simulink model "kinovaMicoSimscapeModel"  (R2021b)
settings: Solver=VariableStepAuto  StartTime=0.0  StopTime=0.3  FixedStep=0.01  RelTol=1e-3
PostLoadFcn:
  | micoRigidBodyTreeCreation;
  | IC=deg2rad([-90,180,180,0,0,0]);
  | interactiveHomePosition=deg2rad([-90 90 177.5 90 0 0]');
  | load("./KinovaMicoSimscapeVariantConfigurations.mat");
values from neighbouring files (symbols this model uses):
  micoCandlePosition = deg2rad([0,180,180,0,0,0])    [KinovaMicoSimscapeInitializeScript.m]    (also in generatingRandomTrajectory.m)
  ViaPointsTaskSpace = [ViaPointsTaskSpace;[[pi;0;pi],[pi;0;pi],[pi;0;pi],[pi;0;pi],[0;0;0],[0;0;0],[pi;0;pi]]]    [KinovaMicoSimscapeInitializeScript.m]    (also in generatingRandomTrajectory.m = [ViaPointsTaskSpace;zeros(3,7)])
undefined symbols (not defined in the file or in its folder): Mico, ViaPointsJointSpace, X, Y, Z
libraries: sm_lib x26, nesl_utility x19, robotcorelib x4, robotmaniplib x3, pid_lib x2
(part 32 of 50)

== matlab function kinovaMicoSimscapeModel/Variant Subsystem/TaskSpaceController/HybridImpedanceVelocityControl/Hybrid Impedance Velocity Control ==
  data: q input; dq input; ddq input; qd input; dqd input; torque output; ddqd input; f input; H input; C input; G input; test output
function [torque,test]     = ImpedanceVelocityControl(q,dq,ddq,qd,dqd,ddqd,f,H,C,G)
%% Joint Space variables
q1 = q(1);
q2 = q(2);
q3 = q(3);
q4 = q(4);
q5 = q(5);
q6 = q(6);

qd1 = qd(1);
qd2 = qd(2);
qd3 = qd(3);
qd4 = qd(4);
qd5 = qd(5);
qd6 = qd(6);


dq1 = qd(1);
dq2 = qd(2);
dq3 = qd(3);
dq4 = qd(4);
dq5 = qd(5);
dq6 = qd(6);


%% Define the Jacobian
jac=[(37*cos(q1)*cos(q4))/1000 - (7*cos(q1))/1000 - (29*sin(q1)*sin(q2))/100 - (37*cos(q5)*(cos(q1)*cos(q4) - sin(q4)*(sin(q1)*sin(q2)*sin(q3) + cos(q2)*cos(q3)*sin(q1))))/2000 + (37*sin(q5)*(cos(q1)*sin(q4) + cos(q4)*(sin(q1)*sin(q2)*sin(q3) + cos(q2)*cos(q3)*sin(q1))))/1000 - (29*3^(1/2)*((cos(q5)*(cos(q1)*cos(q4) - sin(q4)*(sin(q1)*sin(q2)*sin(q3) + cos(q2)*cos(q3)*sin(q1))))/2 - sin(q5)*(cos(q1)*sin(q4) + cos(q4)*(sin(q1)*sin(q2)*sin(q3) + cos(q2)*cos(q3)*sin(q1))) + (3^(1/2)*cos(q5)*(cos(q2)*sin(q1)*sin(q3) - cos(q3)*sin(q1)*sin(q2)))/2))/625 - (37*sin(q4)*(sin(q1)*sin(q2)*sin(q3) + cos(q2)*cos(q3)*sin(q1)))/1000 + (221*3^(1/2)*(cos(q1)*cos(q4) - sin(q4)*(sin(q1)*sin(q2)*sin(q3) + cos(q2)*cos(q3)*sin(q1))))/4000 - (37*3^(1/2)*cos(q5)*(cos(q2)*sin(q1)*sin(q3) - cos(q3)*sin(q1)*sin(q2)))/2000 - (4849*cos(q2)*sin(q1)*sin(q3))/20000 + (4849*cos(q3)*sin(q1)*sin(q2))/20000, (29*cos(q1)*cos(q2))/100 + (37*sin(q4)*(cos(q1)*cos(q2)*sin(q3) - cos(q1)*cos(q3)*sin(q2)))/1000 - (29*3^(1/2)*(cos(q4)*sin(q5)*(cos(q1)*cos(q2)*sin(q3) - cos(q1)*cos(q3)*sin(q2)) + (cos(q5)*sin(q4)*(cos(q1)*cos(q2)*sin(q3) - cos(q1)*cos(q3)*sin(q2)))/2 + (3^(1/2)*cos(q5)*(cos(q1)*cos(q2)*cos(q3) + cos(q1)*sin(q2)*sin(q3)))/2))/625 - (37*cos(q4)*sin(q5)*(cos(q1)*cos(q2)*sin(q3) - cos(q1)*cos(q3)*sin(q2)))/1000 - (37*cos(q5)*sin(q4)*(cos(q1)*cos(q2)*sin(q3) - cos(q1)*cos(q3)*sin(q2)))/2000 - (37*3^(1/2)*cos(q5)*(cos(q1)*cos(q2)*cos(q3) + cos(q1)*sin(q2)*sin(q3)))/2000 + (221*3^(1/2)*sin(q4)*(cos(q1)*cos(q2)*sin(q3) - cos(q1)*cos(q3)*sin(q2)))/4000 - (4849*cos(q1)*cos(q2)*cos(q3))/20000 - (4849*cos(q1)*sin(q2)*sin(q3))/20000, (29*3^(1/2)*(cos(q4)*sin(q5)*(cos(q1)*cos(q2)*sin(q3) - cos(q1)*cos(q3)*sin(q2)) + (cos(q5)*sin(q4)*(cos(q1)*cos(q2)*sin(q3) - cos(q1)*cos(q3)*sin(q2)))/2 + (3^(1/2)*cos(q5)*(cos(q1)*cos(q2)*cos(q3) + cos(q1)*sin(q2)*sin(q3)))/2))/625 - (37*sin(q4)*(cos(q1)*cos(q2)*sin(q3) - cos(q1)*cos(q3)*sin(q2)))/1000 + (37*cos(q4)*sin(q5)*(cos(q1)*cos(q2)*sin(q3) - cos(q1)*cos(q3)*sin(q2)))/1000 + (37*cos(q5)*sin(q4)*(cos(q1)*cos(q2)*sin(q3) - cos(q1)*cos(q3)*sin(q2)))/2000 + (37*3^(1/2)*cos(q5)*(cos(q1)*cos(q2)*cos(q3) + cos(q1)*sin(q2)*sin(q3)))/2000 - (221*3^(1/2)*sin(q4)*(cos(q1)*cos(q2)*sin(q3) - cos(q1)*cos(q3)*sin(q2)))/4000 + (4849*cos(q1)*cos(q2)*cos(q3))/20000 + (4849*cos(q1)*sin(q2)*sin(q3))/20000, (37*cos(q5)*(sin(q1)*sin(q4) - cos(q4)*(cos(q1)*cos(q2)*cos(q3) + cos(q1)*sin(q2)*sin(q3))))/2000 - (37*sin(q1)*sin(q4))/1000 + (37*sin(q5)*(cos(q4)*sin(q1) + sin(q4)*(cos(q1)*cos(q2)*cos(q3) + cos(q1)*sin(q2)*sin(q3))))/1000 + (37*cos(q4)*(cos(q1)*cos(q2)*cos(q3) + cos(q1)*sin(q2)*sin(q3)))/1000 + (29*3^(1/2)*((cos(q5)*(sin(q1)*sin(q4) - cos(q4)*(cos(q1)*cos(q2)*cos(q3) + cos(q1)*sin(q2)*sin(q3))))/2 + sin(q5)*(cos(q4)*sin(q1) + sin(q4)*(cos(q1)*cos(q2)*cos(q3) + cos(q1)*sin(q2)*sin(q3)))))/625 - (221*3^(1/2)*(sin(q1)*sin(q4) - cos(q4)*(cos(q1)*cos(q2)*cos(q3) + cos(q1)*sin(q2)*sin(q3))))/4000, (37*cos(q5)*(sin(q1)*sin(q4) - cos(q4)*(cos(q1)*cos(q2)*cos(q3) + cos(q1)*sin(q2)*sin(q3))))/1000 + (37*sin(q5)*(cos(q4)*sin(q1) + sin(q4)*(cos(q1)*cos(q2)*cos(q3) + cos(q1)*sin(q2)*sin(q3))))/2000 + (29*3^(1/2)*(cos(q5)*(sin(q1)*sin(q4) - cos(q4)*(cos(q1)*cos(q2)*cos(q3) + cos(q1)*sin(q2)*sin(q3))) + (sin(q5)*(cos(q4)*sin(q1) + sin(q4)*(cos(q1)*cos(q2)*cos(q3) + cos(q1)*sin(q2)*sin(q3))))/2 - (3^(1/2)*sin(q5)*(cos(q1)*cos(q2)*sin(q3) - cos(q1)*cos(q3)*sin(q2)))/2))/625 - (37*3^(1/2)*sin(q5)*(cos(q1)*cos(q2)*sin(q3) - cos(q1)*cos(q3)*sin(q2)))/2000,                                                                                                                                                                                                                                                                                                                                                                                                                                       0;
(7*sin(q1))/1000 - (29*cos(q1)*sin(q2))/100 - (37*cos(q4)*sin(q1))/1000 + (37*cos(q5)*(cos(q4)*sin(q1) + sin(q4)*(cos(q1)*cos(q2)*cos(q3) + cos(q1)*sin(q2)*sin(q3))))/2000 - (37*sin(q5)*(sin(q1)*sin(q4) - cos(q4)*(cos(q1)*cos(q2)*cos(q3) + cos(q1)*sin(q2)*sin(q3))))/1000 - (29*3^(1/2)*(sin(q5)*(sin(q1)*sin(q4) - cos(q4)*(cos(q1)*cos(q2)*cos(q3) + cos(q1)*sin(q2)*sin(q3))) - (cos(q5)*(cos(q4)*sin(q1) + sin(q4)*(cos(q1)*cos(q2)*cos(q3) + cos(q1)*sin(q2)*sin(q3))))/2 + (3^(1/2)*cos(q5)*(cos(q1)*cos(q2)*sin(q3) - cos(q1)*cos(q3)*sin(q2)))/2))/625 - (37*sin(q4)*(cos(q1)*cos(q2)*cos(q3) + cos(q1)*sin(q2)*sin(q3)))/1000 - (221*3^(1/2)*(cos(q4)*sin(q1) + sin(q4)*(cos(q1)*cos(q2)*cos(q3) + cos(q1)*sin(q2)*sin(q3))))/4000 - (37*3^(1/2)*cos(q5)*(cos(q1)*cos(q2)*sin(q3) - cos(q1)*cos(q3)*sin(q2)))/2000 - (4849*cos(q1)*cos(q2)*sin(q3))/20000 + (4849*cos(q1)*cos(q3)*sin(q2))/20000, (29*3^(1/2)*(cos(q4)*sin(q5)*(cos(q2)*sin(q1)*sin(q3) - cos(q3)*sin(q1)*sin(q2)) + (cos(q5)*sin(q4)*(cos(q2)*sin(q1)*sin(q3) - cos(q3)*sin(q1)*sin(q2)))/2 + (3^(1/2)*cos(q5)*(sin(q1)*sin(q2)*sin(q3) + cos(q2)*cos(q3)*sin(q1)))/2))/625 - (37*sin(q4)*(cos(q2)*sin(q1)*sin(q3) - cos(q3)*sin(q1)*sin(q2)))/1000 - (29*cos(q2)*sin(q1))/100 + (4849*sin(q1)*sin(q2)*sin(q3))/20000 + (37*cos(q4)*sin(q5)*(cos(q2)*sin(q1)*sin(q3) - cos(q3)*sin(q1)*sin(q2)))/1000 + (37*cos(q5)*sin(q4)*(cos(q2)*sin(q1)*sin(q3) - cos(q3)*sin(q1)*sin(q2)))/2000 + (37*3^(1/2)*cos(q5)*(sin(q1)*sin(q2)*sin(q3) + cos(q2)*cos(q3)*sin(q1)))/2000 + (4849*cos(q2)*cos(q3)*sin(q1))/20000 - (221*3^(1/2)*sin(q4)*(cos(q2)*sin(q1)*sin(q3) - cos(q3)*sin(q1)*sin(q2)))/4000, (37*sin(q4)*(cos(q2)*sin(q1)*sin(q3) - cos(q3)*sin(q1)*sin(q2)))/1000 - (29*3^(1/2)*(cos(q4)*sin(q5)*(cos(q2)*sin(q1)*sin(q3) - cos(q3)*sin(q1)*sin(q2)) + (cos(q5)*sin(q4)*(cos(q2)*sin(q1)*sin(q3) - cos(q3)*sin(q1)*sin(q2)))/2 + (3^(1/2)*cos(q5)*(sin(q1)*sin(q2)*sin(q3) + cos(q2)*cos(q3)*sin(q1)))/2))/625 - (4849*sin(q1)*sin(q2)*sin(q3))/20000 - (37*cos(q4)*sin(q5)*(cos(q2)*sin(q1)*sin(q3) - cos(q3)*sin(q1)*sin(q2)))/1000 - (37*cos(q5)*sin(q4)*(cos(q2)*sin(q1)*sin(q3) - cos(q3)*sin(q1)*sin(q2)))/2000 - (37*3^(1/2)*cos(q5)*(sin(q1)*sin(q2)*sin(q3) + cos(q2)*cos(q3)*sin(q1)))/2000 - (4849*cos(q2)*cos(q3)*sin(q1))/20000 + (221*3^(1/2)*sin(q4)*(cos(q2)*sin(q1)*sin(q3) - cos(q3)*sin(q1)*sin(q2)))/4000, (37*cos(q5)*(cos(q1)*sin(q4) + cos(q4)*(sin(q1)*sin(q2)*sin(q3) + cos(q2)*cos(q3)*sin(q1))))/2000 - (37*cos(q1)*sin(q4))/1000 + (37*sin(q5)*(cos(q1)*cos(q4) - sin(q4)*(sin(q1)*sin(q2)*sin(q3) + cos(q2)*cos(q3)*sin(q1))))/1000 - (37*cos(q4)*(sin(q1)*sin(q2)*sin(q3) + cos(q2)*cos(q3)*sin(q1)))/1000 + (29*3^(1/2)*((cos(q5)*(cos(q1)*sin(q4) + cos(q4)*(sin(q1)*sin(q2)*sin(q3) + cos(q2)*cos(q3)*sin(q1))))/2 + sin(q5)*(cos(q1)*cos(q4) - sin(q4)*(sin(q1)*sin(q2)*sin(q3) + cos(q2)*cos(q3)*sin(q1)))))/625 - (221*3^(1/2)*(cos(q1)*sin(q4) + cos(q4)*(sin(q1)*sin(q2)*sin(q3) + cos(q2)*cos(q3)*sin(q1))))/4000, (37*cos(q5)*(cos(q1)*sin(q4) + cos(q4)*(sin(q1)*sin(q2)*sin(q3) + cos(q2)*cos(q3)*sin(q1))))/1000 + (37*sin(q5)*(cos(q1)*cos(q4) - sin(q4)*(sin(q1)*sin(q2)*sin(q3) + cos(q2)*cos(q3)*sin(q1))))/2000 + (29*3^(1/2)*(cos(q5)*(cos(q1)*sin(q4) + cos(q4)*(sin(q1)*sin(q2)*sin(q3) + cos(q2)*cos(q3)*sin(q1))) + (sin(q5)*(cos(q1)*cos(q4) - sin(q4)*(sin(q1)*sin(q2)*sin(q3) + cos(q2)*cos(q3)*sin(q1))))/2 + (3^(1/2)*sin(q5)*(cos(q2)*sin(q1)*sin(q3) - cos(q3)*sin(q1)*sin(q2)))/2))/625 + (37*3^(1/2)*sin(q5)*(cos(q2)*sin(q1)*sin(q3) - cos(q3)*sin(q1)*sin(q2)))/2000,                                                                                                                                                                                                                                                                                                                                                                                                                                       0;
                                                                                                                                                                                                                                                                                                                                                                                                                                                                                                                                                                                                                                                                                                                                                                                                                                                                                                              0,                                                                                                                                                         (29*sin(q2))/100 + (4849*cos(q2)*sin(q3))/20000 - (4849*cos(q3)*sin(q2))/20000 - (29*3^(1/2)*(cos(q4)*sin(q5)*(cos(q2)*cos(q3) + sin(q2)*sin(q3)) - (3^(1/2)*cos(q5)*(cos(q2)*sin(q3) - cos(q3)*sin(q2)))/2 + (cos(q5)*sin(q4)*(cos(q2)*cos(q3) + sin(q2)*sin(q3)))/2))/625 + (37*sin(q4)*(cos(q2)*cos(q3) + sin(q2)*sin(q3)))/1000 + (37*3^(1/2)*cos(q5)*(cos(q2)*sin(q3) - cos(q3)*sin(q2)))/2000 + (221*3^(1/2)*sin(q4)*(cos(q2)*cos(q3) + sin(q2)*sin(q3)))/4000 - (37*cos(q4)*sin(q5)*(cos(q2)*cos(q3) + sin(q2)*sin(q3)))/1000 - (37*cos(q5)*sin(q4)*(cos(q2)*cos(q3) + sin(q2)*sin(q3)))/2000,                                                                                                                                                 (4849*cos(q3)*sin(q2))/20000 - (4849*cos(q2)*sin(q3))/20000 + (29*3^(1/2)*(cos(q4)*sin(q5)*(cos(q2)*cos(q3) + sin(q2)*sin(q3)) - (3^(1/2)*cos(q5)*(cos(q2)*sin(q3) - cos(q3)*sin(q2)))/2 + (cos(q5)*sin(q4)*(cos(q2)*cos(q3) + sin(q2)*sin(q3)))/2))/625 - (37*sin(q4)*(cos(q2)*cos(q3) + sin(q2)*sin(q3)))/1000 - (37*3^(1/2)*cos(q5)*(cos(q2)*sin(q3) - cos(q3)*sin(q2)))/2000 - (221*3^(1/2)*sin(q4)*(cos(q2)*cos(q3) + sin(q2)*sin(q3)))/4000 + (37*cos(q4)*sin(q5)*(cos(q2)*cos(q3) + sin(q2)*sin(q3)))/1000 + (37*cos(q5)*sin(q4)*(cos(q2)*cos(q3) + sin(q2)*sin(q3)))/2000,                                                                                                                                                                                                                                 (29*3^(1/2)*((cos(q4)*cos(q5)*(cos(q2)*sin(q3) - cos(q3)*sin(q2)))/2 - sin(q4)*sin(q5)*(cos(q2)*sin(q3) - cos(q3)*sin(q2))))/625 - (37*cos(q4)*(cos(q2)*sin(q3) - cos(q3)*sin(q2)))/1000 - (221*3^(1/2)*cos(q4)*(cos(q2)*sin(q3) - cos(q3)*sin(q2)))/4000 + (37*cos(q4)*cos(q5)*(cos(q2)*sin(q3) - cos(q3)*sin(q2)))/2000 - (37*sin(q4)*sin(q5)*(cos(q2)*sin(q3) - cos(q3)*sin(q2)))/1000,                                                                                                                                                                                 (37*cos(q4)*cos(q5)*(cos(q2)*sin(q3) - cos(q3)*sin(q2)))/1000 - (37*3^(1/2)*sin(q5)*(cos(q2)*cos(q3) + sin(q2)*sin(q3)))/2000 - (29*3^(1/2)*((3^(1/2)*sin(q5)*(cos(q2)*cos(q3) + sin(q2)*sin(q3)))/2 - cos(q4)*cos(q5)*(cos(q2)*sin(q3) - cos(q3)*sin(q2)) + (sin(q4)*sin(q5)*(cos(q2)*sin(q3) - cos(q3)*sin(q2)))/2))/625 - (37*sin(q4)*sin(q5)*(cos(q2)*sin(q3) - cos(q3)*sin(q2)))/2000,                                                                                                                                                                                                                                                                                                                                                                                                                                       0;
                                                                                                                                                                                                                                                                                                                                                                                                                                                                                                                                                                                                                                                                                                                                                                                                                                                                                                              0,                                                                                                                                                                                                                                                                                                                                                                                                                                                                                                                                                                                                                                                                                                                                                     -sin(q1),                                                                                                                                                                                                                                                                                                                                                                                                                                                                                                                                                                                                                                                                                                                           sin(q1),                                                                                                                                                                                                                                                                                                                                                                                                                                                                                                                                                                         cos(q1)*cos(q3)*sin(q2) - cos(q1)*cos(q2)*sin(q3),                                                                                                                                                                                                                                                                                                                                                                                                                    (cos(q1)*cos(q3)*sin(q2))/2 - (cos(q1)*cos(q2)*sin(q3))/2 - (3^(1/2)*(cos(q4)*sin(q1) + sin(q4)*(cos(q1)*cos(q2)*cos(q3) + cos(q1)*sin(q2)*sin(q3))))/2, (cos(q1)*cos(q3)*sin(q2))/4 - (3^(1/2)*(cos(q4)*sin(q1) + sin(q4)*(cos(q1)*cos(q2)*cos(q3) + cos(q1)*sin(q2)*sin(q3))))/4 - (cos(q1)*cos(q2)*sin(q3))/4 - (3^(1/2)*(sin(q5)*(sin(q1)*sin(q4) - cos(q4)*(cos(q1)*cos(q2)*cos(q3) + cos(q1)*sin(q2)*sin(q3))) - (cos(q5)*(cos(q4)*sin(q1) + sin(q4)*(cos(q1)*cos(q2)*cos(q3) + cos(q1)*sin(q2)*sin(q3))))/2 + (3^(1/2)*cos(q5)*(cos(q1)*cos(q2)*sin(q3) - cos(q1)*cos(q3)*sin(q2)))/2))/2;
                                                                                                                                                                                                                                                                                                                                                                                                                                                                                                                                                                                                                                                                                                                                                                                                                                                                                                              0,                                                                                                                                                                                                                                                                                                                                                                                                                                                                                                                                                                                                                                                                                                                                                     -cos(q1),                                                                                                                                                                                                                                                                                                                                                                                                                                                                                                                                                                                                                                                                                                                           cos(q1),                                                                                                                                                                                                                                                                                                                                                                                                                                                                                                                                                                         cos(q2)*sin(q1)*sin(q3) - cos(q3)*sin(q1)*sin(q2),                                                                                                                                                                                                                                                                                                                                                                                                                    (cos(q2)*sin(q1)*sin(q3))/2 - (3^(1/2)*(cos(q1)*cos(q4) - sin(q4)*(sin(q1)*sin(q2)*sin(q3) + cos(q2)*cos(q3)*sin(q1))))/2 - (cos(q3)*sin(q1)*sin(q2))/2, (3^(1/2)*((cos(q5)*(cos(q1)*cos(q4) - sin(q4)*(sin(q1)*sin(q2)*sin(q3) + cos(q2)*cos(q3)*sin(q1))))/2 - sin(q5)*(cos(q1)*sin(q4) + cos(q4)*(sin(q1)*sin(q2)*sin(q3) + cos(q2)*cos(q3)*sin(q1))) + (3^(1/2)*cos(q5)*(cos(q2)*sin(q1)*sin(q3) - cos(q3)*sin(q1)*sin(q2)))/2))/2 - (3^(1/2)*(cos(q1)*cos(q4) - sin(q4)*(sin(q1)*sin(q2)*sin(q3) + cos(q2)*cos(q3)*sin(q1))))/4 + (cos(q2)*sin(q1)*sin(q3))/4 - (cos(q3)*sin(q1)*sin(q2))/4;
                                                                                                                                                                                                                                                                                                                                                                                                                                                                                                                                                                                                                                                                                                                                                                                                                                                                                                             -1,                                                                                                                                                                                                                                                                                                                                                                                                                                                                                                                                                                                                                                                                                                                                                            0,                                                                                                                                                                                                                                                                                                                                                                                                                                                                                                                                                                                                                                                                                                                                 0,                                                                                                                                                                                                                                                                                                                                                                                                                                                                                                                                                                                       - cos(q2)*cos(q3) - sin(q2)*sin(q3),                                                                                                                                                                                                                                                                                                                                                                                                                                                                        (3^(1/2)*sin(q4)*(cos(q2)*sin(q3) - cos(q3)*sin(q2)))/2 - (sin(q2)*sin(q3))/2 - (cos(q2)*cos(q3))/2,                                                                                                                                             (3^(1/2)*sin(q4)*(cos(q2)*sin(q3) - cos(q3)*sin(q2)))/4 - (sin(q2)*sin(q3))/4 - (3^(1/2)*((3^(1/2)*cos(q5)*(cos(q2)*cos(q3) + sin(q2)*sin(q3)))/2 + cos(q4)*sin(q5)*(cos(q2)*sin(q3) - cos(q3)*sin(q2)) + (cos(q5)*sin(q4)*(cos(q2)*sin(q3) - cos(q3)*sin(q2)))/2))/2 - (cos(q2)*cos(q3))/4];
                        
%% Define the derivative of the jacobian
dJac=[(37*cos(q5)*(sin(q4)*(dq1*cos(q1)*cos(q2)*cos(q3) + dq1*cos(q1)*sin(q2)*sin(q3) + dq2*cos(q2)*sin(q1)*sin(q3) - dq2*cos(q3)*sin(q1)*sin(q2) - dq3*cos(q2)*sin(q1)*sin(q3) + dq3*cos(q3)*sin(q1)*sin(q2)) + dq1*cos(q4)*sin(q1) + dq4*cos(q1)*sin(q4) + dq4*cos(q4)*(sin(q1)*sin(q2)*sin(q3) + cos(q2)*cos(q3)*sin(q1))))/2000 + (37*sin(q5)*(cos(q4)*(dq1*cos(q1)*cos(q2)*cos(q3) + dq1*cos(q1)*sin(q2)*sin(q3) + dq2*cos(q2)*sin(q1)*sin(q3) - dq2*cos(q3)*sin(q1)*sin(q2) - dq3*cos(q2)*sin(q1)*sin(q3) + dq3*cos(q3)*sin(q1)*sin(q2)) - dq4*sin(q4)*(sin(q1)*sin(q2)*sin(q3) + cos(q2)*cos(q3)*sin(q1)) + dq4*cos(q1)*cos(q4) - dq1*sin(q1)*sin(q4)))/1000 + (29*3^(1/2)*((cos(q5)*(sin(q4)*(dq1*cos(q1)*cos(q2)*cos(q3) + dq1*cos(q1)*sin(q2)*sin(q3) + dq2*cos(q2)*sin(q1)*sin(q3) - dq2*cos(q3)*sin(q1)*sin(q2) - dq3*cos(q2)*sin(q1)*sin(q3) + dq3*cos(q3)*sin(q1)*sin(q2)) + dq1*cos(q4)*sin(q1) + dq4*cos(q1)*sin(q4) + dq4*cos(q4)*(sin(q1)*sin(q2)*sin(q3) + cos(q2)*cos(q3)*sin(q1))))/2 + sin(q5)*(cos(q4)*(dq1*cos(q1)*cos(q2)*cos(q3) + dq1*cos(q1)*sin(q2)*sin(q3) + dq2*cos(q2)*sin(q1)*sin(q3) - dq2*cos(q3)*sin(q1)*sin(q2) - dq3*cos(q2)*sin(q1)*sin(q3) + dq3*cos(q3)*sin(q1)*sin(q2)) - dq4*sin(q4)*(sin(q1)*sin(q2)*sin(q3) + cos(q2)*cos(q3)*sin(q1)) + dq4*cos(q1)*cos(q4) - dq1*sin(q1)*sin(q4)) - (3^(1/2)*cos(q5)*(dq1*cos(q1)*cos(q2)*sin(q3) - dq1*cos(q1)*cos(q3)*sin(q2) - dq2*cos(q2)*cos(q3)*sin(q1) + dq3*cos(q2)*cos(q3)*sin(q1) - dq2*sin(q1)*sin(q2)*sin(q3) + dq3*sin(q1)*sin(q2)*sin(q3)))/2 + dq5*cos(q5)*(cos(q1)*sin(q4) + cos(q4)*(sin(q1)*sin(q2)*sin(q3) + cos(q2)*cos(q3)*sin(q1))) + (dq5*sin(q5)*(cos(q1)*cos(q4) - sin(q4)*(sin(q1)*sin(q2)*sin(q3) + cos(q2)*cos(q3)*sin(q1))))/2 + (3^(1/2)*dq5*sin(q5)*(cos(q2)*sin(q1)*sin(q3) - cos(q3)*sin(q1)*sin(q2)))/2))/625 + (7*dq1*sin(q1))/1000 - (37*sin(q4)*(dq1*cos(q1)*cos(q2)*cos(q3) + dq1*cos(q1)*sin(q2)*sin(q3) + dq2*cos(q2)*sin(q1)*sin(q3) - dq2*cos(q3)*sin(q1)*sin(q2) - dq3*cos(q2)*sin(q1)*sin(q3) + dq3*cos(q3)*sin(q1)*sin(q2)))/1000 - (221*3^(1/2)*(sin(q4)*(dq1*cos(q1)*cos(q2)*cos(q3) + dq1*cos(q1)*sin(q2)*sin(q3) + dq2*cos(q2)*sin(q1)*sin(q3) - dq2*cos(q3)*sin(q1)*sin(q2) - dq3*cos(q2)*sin(q1)*sin(q3) + dq3*cos(q3)*sin(q1)*sin(q2)) + dq1*cos(q4)*sin(q1) + dq4*cos(q1)*sin(q4) + dq4*cos(q4)*(sin(q1)*sin(q2)*sin(q3) + cos(q2)*cos(q3)*sin(q1))))/4000 - (37*3^(1/2)*cos(q5)*(dq1*cos(q1)*cos(q2)*sin(q3) - dq1*cos(q1)*cos(q3)*sin(q2) - dq2*cos(q2)*cos(q3)*sin(q1) + dq3*cos(q2)*cos(q3)*sin(q1) - dq2*sin(q1)*sin(q2)*sin(q3) + dq3*sin(q1)*sin(q2)*sin(q3)))/2000 - (29*dq1*cos(q1)*sin(q2))/100 - (29*dq2*cos(q2)*sin(q1))/100 - (37*dq1*cos(q4)*sin(q1))/1000 - (37*dq4*cos(q1)*sin(q4))/1000 + (37*dq5*cos(q5)*(cos(q1)*sin(q4) + cos(q4)*(sin(q1)*sin(q2)*sin(q3) + cos(q2)*cos(q3)*sin(q1))))/1000 + (37*dq5*sin(q5)*(cos(q1)*cos(q4) - sin(q4)*(sin(q1)*sin(q2)*sin(q3) + cos(q2)*cos(q3)*sin(q1))))/2000 - (37*dq4*cos(q4)*(sin(q1)*sin(q2)*sin(q3) + cos(q2)*cos(q3)*sin(q1)))/1000 - (4849*dq1*cos(q1)*cos(q2)*sin(q3))/20000 + (4849*dq1*cos(q1)*cos(q3)*sin(q2))/20000 + (4849*dq2*cos(q2)*cos(q3)*sin(q1))/20000 - (4849*dq3*cos(q2)*cos(q3)*sin(q1))/20000 + (37*3^(1/2)*dq5*sin(q5)*(cos(q2)*sin(q1)*sin(q3) - cos(q3)*sin(q1)*sin(q2)))/2000 + (4849*dq2*sin(q1)*sin(q2)*sin(q3))/20000 - (4849*dq3*sin(q1)*sin(q2)*sin(q3))/20000, (29*3^(1/2)*(cos(q4)*sin(q5)*(dq2*cos(q1)*cos(q2)*cos(q3) - dq3*cos(q1)*cos(q2)*cos(q3) + dq1*cos(q2)*sin(q1)*sin(q3) - dq1*cos(q3)*sin(q1)*sin(q2) + dq2*cos(q1)*sin(q2)*sin(q3) - dq3*cos(q1)*sin(q2)*sin(q3)) + (cos(q5)*sin(q4)*(dq2*cos(q1)*cos(q2)*cos(q3) - dq3*cos(q1)*cos(q2)*cos(q3) + dq1*cos(q2)*sin(q1)*sin(q3) - dq1*cos(q3)*sin(q1)*sin(q2) + dq2*cos(q1)*sin(q2)*sin(q3) - dq3*cos(q1)*sin(q2)*sin(q3)))/2 + (3^(1/2)*cos(q5)*(dq1*cos(q2)*cos(q3)*sin(q1) - dq2*cos(q1)*cos(q2)*sin(q3) + dq2*cos(q1)*cos(q3)*sin(q2) + dq3*cos(q1)*cos(q2)*sin(q3) - dq3*cos(q1)*cos(q3)*sin(q2) + dq1*sin(q1)*sin(q2)*sin(q3)))/2 + (3^(1/2)*dq5*sin(q5)*(cos(q1)*cos(q2)*cos(q3) + cos(q1)*sin(q2)*sin(q3)))/2 - (dq4*cos(q4)*cos(q5)*(cos(q1)*cos(q2)*sin(q3) - cos(q1)*cos(q3)*sin(q2)))/2 - dq5*cos(q4)*cos(q5)*(cos(q1)*cos(q2)*sin(q3) - cos(q1)*cos(q3)*sin(q2)) + dq4*sin(q4)*sin(q5)*(cos(q1)*cos(q2)*sin(q3) - cos(q1)*cos(q3)*sin(q2)) + (dq5*sin(q4)*sin(q5)*(cos(q1)*cos(q2)*sin(q3) - cos(q1)*cos(q3)*sin(q2)))/2))/625 - (37*sin(q4)*(dq2*cos(q1)*cos(q2)*cos(q3) - dq3*cos(q1)*cos(q2)*cos(q3) + dq1*cos(q2)*sin(q1)*sin(q3) - dq1*cos(q3)*sin(q1)*sin(q2) + dq2*cos(q1)*sin(q2)*sin(q3) - dq3*cos(q1)*sin(q2)*sin(q3)))/1000 - (221*3^(1/2)*sin(q4)*(dq2*cos(q1)*cos(q2)*cos(q3) - dq3*cos(q1)*cos(q2)*cos(q3) + dq1*cos(q2)*sin(q1)*sin(q3) - dq1*cos(q3)*sin(q1)*sin(q2) + dq2*cos(q1)*sin(q2)*sin(q3) - dq3*cos(q1)*sin(q2)*sin(q3)))/4000 - (29*dq1*cos(q2)*sin(q1))/100 - (29*dq2*cos(q1)*sin(q2))/100 + (37*cos(q4)*sin(q5)*(dq2*cos(q1)*cos(q2)*cos(q3) - dq3*cos(q1)*cos(q2)*cos(q3) + dq1*cos(q2)*sin(q1)*sin(q3) - dq1*cos(q3)*sin(q1)*sin(q2) + dq2*cos(q1)*sin(q2)*sin(q3) - dq3*cos(q1)*sin(q2)*sin(q3)))/1000 + (37*cos(q5)*sin(q4)*(dq2*cos(q1)*cos(q2)*cos(q3) - dq3*cos(q1)*cos(q2)*cos(q3) + dq1*cos(q2)*sin(q1)*sin(q3) - dq1*cos(q3)*sin(q1)*sin(q2) + dq2*cos(q1)*sin(q2)*sin(q3) - dq3*cos(q1)*sin(q2)*sin(q3)))/2000 + (37*dq4*cos(q4)*(cos(q1)*cos(q2)*sin(q3) - cos(q1)*cos(q3)*sin(q2)))/1000 + (37*3^(1/2)*cos(q5)*(dq1*cos(q2)*cos(q3)*sin(q1) - dq2*cos(q1)*cos(q2)*sin(q3) + dq2*cos(q1)*cos(q3)*sin(q2) + dq3*cos(q1)*cos(q2)*sin(q3) - dq3*cos(q1)*cos(q3)*sin(q2) + dq1*sin(q1)*sin(q2)*sin(q3)))/2000 + (221*3^(1/2)*dq4*cos(q4)*(cos(q1)*cos(q2)*sin(q3) - cos(q1)*cos(q3)*sin(q2)))/4000 + (37*3^(1/2)*dq5*sin(q5)*(cos(q1)*cos(q2)*cos(q3) + cos(q1)*sin(q2)*sin(q3)))/2000 + (4849*dq1*cos(q2)*cos(q3)*sin(q1))/20000 - (4849*dq2*cos(q1)*cos(q2)*sin(q3))/20000 + (4849*dq2*cos(q1)*cos(q3)*sin(q2))/20000 + (4849*dq3*cos(q1)*cos(q2)*sin(q3))/20000 - (4849*dq3*cos(q1)*cos(q3)*sin(q2))/20000 + (4849*dq1*sin(q1)*sin(q2)*sin(q3))/20000 - (37*dq4*cos(q4)*cos(q5)*(cos(q1)*cos(q2)*sin(q3) - cos(q1)*cos(q3)*sin(q2)))/2000 - (37*dq5*cos(q4)*cos(q5)*(cos(q1)*cos(q2)*sin(q3) - cos(q1)*cos(q3)*sin(q2)))/1000 + (37*dq4*sin(q4)*sin(q5)*(cos(q1)*cos(q2)*sin(q3) - cos(q1)*cos(q3)*sin(q2)))/1000 + (37*dq5*sin(q4)*sin(q5)*(cos(q1)*cos(q2)*sin(q3) - cos(q1)*cos(q3)*sin(q2)))/2000, (37*sin(q4)*(dq2*cos(q1)*cos(q2)*cos(q3) - dq3*cos(q1)*cos(q2)*cos(q3) + dq1*cos(q2)*sin(q1)*sin(q3) - dq1*cos(q3)*sin(q1)*sin(q2) + dq2*cos(q1)*sin(q2)*sin(q3) - dq3*cos(q1)*sin(q2)*sin(q3)))/1000 - (29*3^(1/2)*(cos(q4)*sin(q5)*(dq2*cos(q1)*cos(q2)*cos(q3) - dq3*cos(q1)*cos(q2)*cos(q3) + dq1*cos(q2)*sin(q1)*sin(q3) - dq1*cos(q3)*sin(q1)*sin(q2) + dq2*cos(q1)*sin(q2)*sin(q3) - dq3*cos(q1)*sin(q2)*sin(q3)) + (cos(q5)*sin(q4)*(dq2*cos(q1)*cos(q2)*cos(q3) - dq3*cos(q1)*cos(q2)*cos(q3) + dq1*cos(q2)*sin(q1)*sin(q3) - dq1*cos(q3)*sin(q1)*sin(q2) + dq2*cos(q1)*sin(q2)*sin(q3) - dq3*cos(q1)*sin(q2)*sin(q3)))/2 + (3^(1/2)*cos(q5)*(dq1*cos(q2)*cos(q3)*sin(q1) - dq2*cos(q1)*cos(q2)*sin(q3) + dq2*cos(q1)*cos(q3)*sin(q2) + dq3*cos(q1)*cos(q2)*sin(q3) - dq3*cos(q1)*cos(q3)*sin(q2) + dq1*sin(q1)*sin(q2)*sin(q3)))/2 + (3^(1/2)*dq5*sin(q5)*(cos(q1)*cos(q2)*cos(q3) + cos(q1)*sin(q2)*sin(q3)))/2 - (dq4*cos(q4)*cos(q5)*(cos(q1)*cos(q2)*sin(q3) - cos(q1)*cos(q3)*sin(q2)))/2 - dq5*cos(q4)*cos(q5)*(cos(q1)*cos(q2)*sin(q3) - cos(q1)*cos(q3)*sin(q2)) + dq4*sin(q4)*sin(q5)*(cos(q1)*cos(q2)*sin(q3) - cos(q1)*cos(q3)*sin(q2)) + (dq5*sin(q4)*sin(q5)*(cos(q1)*cos(q2)*sin(q3) - cos(q1)*cos(q3)*sin(q2)))/2))/625 + (221*3^(1/2)*sin(q4)*(dq2*cos(q1)*cos(q2)*cos(q3) - dq3*cos(q1)*cos(q2)*cos(q3) + dq1*cos(q2)*sin(q1)*sin(q3) - dq1*cos(q3)*sin(q1)*sin(q2) + dq2*cos(q1)*sin(q2)*sin(q3) - dq3*cos(q1)*sin(q2)*sin(q3)))/4000 - (37*cos(q4)*sin(q5)*(dq2*cos(q1)*cos(q2)*cos(q3) - dq3*cos(q1)*cos(q2)*cos(q3) + dq1*cos(q2)*sin(q1)*sin(q3) - dq1*cos(q3)*sin(q1)*sin(q2) + dq2*cos(q1)*sin(q2)*sin(q3) - dq3*cos(q1)*sin(q2)*sin(q3)))/1000 - (37*cos(q5)*sin(q4)*(dq2*cos(q1)*cos(q2)*cos(q3) - dq3*cos(q1)*cos(q2)*cos(q3) + dq1*cos(q2)*sin(q1)*sin(q3) - dq1*cos(q3)*sin(q1)*sin(q2) + dq2*cos(q1)*sin(q2)*sin(q3) - dq3*cos(q1)*sin(q2)*sin(q3)))/2000 - (37*dq4*cos(q4)*(cos(q1)*cos(q2)*sin(q3) - cos(q1)*cos(q3)*sin(q2)))/1000 - (37*3^(1/2)*cos(q5)*(dq1*cos(q2)*cos(q3)*sin(q1) - dq2*cos(q1)*cos(q2)*sin(q3) + dq2*cos(q1)*cos(q3)*sin(q2) + dq3*cos(q1)*cos(q2)*sin(q3) - dq3*cos(q1)*cos(q3)*sin(q2) + dq1*sin(q1)*sin(q2)*sin(q3)))/2000 - (221*3^(1/2)*dq4*cos(q4)*(cos(q1)*cos(q2)*sin(q3) - cos(q1)*cos(q3)*sin(q2)))/4000 - (37*3^(1/2)*dq5*sin(q5)*(cos(q1)*cos(q2)*cos(q3) + cos(q1)*sin(q2)*sin(q3)))/2000 - (4849*dq1*cos(q2)*cos(q3)*sin(q1))/20000 + (4849*dq2*cos(q1)*cos(q2)*sin(q3))/20000 - (4849*dq2*cos(q1)*cos(q3)*sin(q2))/20000 - (4849*dq3*cos(q1)*cos(q2)*sin(q3))/20000 + (4849*dq3*cos(q1)*cos(q3)*sin(q2))/20000 - (4849*dq1*sin(q1)*sin(q2)*sin(q3))/20000 + (37*dq4*cos(q4)*cos(q5)*(cos(q1)*cos(q2)*sin(q3) - cos(q1)*cos(q3)*sin(q2)))/2000 + (37*dq5*cos(q4)*cos(q5)*(cos(q1)*cos(q2)*sin(q3) - cos(q1)*cos(q3)*sin(q2)))/1000 - (37*dq4*sin(q4)*sin(q5)*(cos(q1)*cos(q2)*sin(q3) - cos(q1)*cos(q3)*sin(q2)))/1000 - (37*dq5*sin(q4)*sin(q5)*(cos(q1)*cos(q2)*sin(q3) - cos(q1)*cos(q3)*sin(q2)))/2000, (37*cos(q5)*(cos(q4)*(dq1*cos(q2)*cos(q3)*sin(q1) - dq2*cos(q1)*cos(q2)*sin(q3) + dq2*cos(q1)*cos(q3)*sin(q2) + dq3*cos(q1)*cos(q2)*sin(q3) - dq3*cos(q1)*cos(q3)*sin(q2) + dq1*sin(q1)*sin(q2)*sin(q3)) + dq1*cos(q1)*sin(q4) + dq4*cos(q4)*sin(q1) + dq4*sin(q4)*(cos(q1)*cos(q2)*cos(q3) + cos(q1)*sin(q2)*sin(q3))))/2000 - (37*sin(q5)*(sin(q4)*(dq1*cos(q2)*cos(q3)*sin(q1) - dq2*cos(q1)*cos(q2)*sin(q3) + dq2*cos(q1)*cos(q3)*sin(q2) + dq3*cos(q1)*cos(q2)*sin(q3) - dq3*cos(q1)*cos(q3)*sin(q2) + dq1*sin(q1)*sin(q2)*sin(q3)) - dq1*cos(q1)*cos(q4) + dq4*sin(q1)*sin(q4) - dq4*cos(q4)*(cos(q1)*cos(q2)*cos(q3) + cos(q1)*sin(q2)*sin(q3))))/1000 + (29*3^(1/2)*((cos(q5)*(cos(q4)*(dq1*cos(q2)*cos(q3)*sin(q1) - dq2*cos(q1)*cos(q2)*sin(q3) + dq2*cos(q1)*cos(q3)*sin(q2) + dq3*cos(q1)*cos(q2)*sin(q3) - dq3*cos(q1)*cos(q3)*sin(q2) + dq1*sin(q1)*sin(q2)*sin(q3)) + dq1*cos(q1)*sin(q4) + dq4*cos(q4)*sin(q1) + dq4*sin(q4)*(cos(q1)*cos(q2)*cos(q3) + cos(q1)*sin(q2)*sin(q3))))/2 - sin(q5)*(sin(q4)*(dq1*cos(q2)*cos(q3)*sin(q1) - dq2*cos(q1)*cos(q2)*sin(q3) + dq2*cos(q1)*cos(q3)*sin(q2) + dq3*cos(q1)*cos(q2)*sin(q3) - dq3*cos(q1)*cos(q3)*sin(q2) + dq1*sin(q1)*sin(q2)*sin(q3)) - dq1*cos(q1)*cos(q4) + dq4*sin(q1)*sin(q4) - dq4*cos(q4)*(cos(q1)*cos(q2)*cos(q3) + cos(q1)*sin(q2)*sin(q3))) + dq5*cos(q5)*(cos(q4)*sin(q1) + sin(q4)*(cos(q1)*cos(q2)*cos(q3) + cos(q1)*sin(q2)*sin(q3))) - (dq5*sin(q5)*(sin(q1)*sin(q4) - cos(q4)*(cos(q1)*cos(q2)*cos(q3) + cos(q1)*sin(q2)*sin(q3))))/2))/625 - (221*3^(1/2)*(cos(q4)*(dq1*cos(q2)*cos(q3)*sin(q1) - dq2*cos(q1)*cos(q2)*sin(q3) + dq2*cos(q1)*cos(q3)*sin(q2) + dq3*cos(q1)*cos(q2)*sin(q3) - dq3*cos(q1)*cos(q3)*sin(q2) + dq1*sin(q1)*sin(q2)*sin(q3)) + dq1*cos(q1)*sin(q4) + dq4*cos(q4)*sin(q1) + dq4*sin(q4)*(cos(q1)*cos(q2)*cos(q3) + cos(q1)*sin(q2)*sin(q3))))/4000 - (37*cos(q4)*(dq1*cos(q2)*cos(q3)*sin(q1) - dq2*cos(q1)*cos(q2)*sin(q3) + dq2*cos(q1)*cos(q3)*sin(q2) + dq3*cos(q1)*cos(q2)*sin(q3) - dq3*cos(q1)*cos(q3)*sin(q2) + dq1*sin(q1)*sin(q2)*sin(q3)))/1000 - (37*dq1*cos(q1)*sin(q4))/1000 - (37*dq4*cos(q4)*sin(q1))/1000 + (37*dq5*cos(q5)*(cos(q4)*sin(q1) + sin(q4)*(cos(q1)*cos(q2)*cos(q3) + cos(q1)*sin(q2)*sin(q3))))/1000 - (37*dq5*sin(q5)*(sin(q1)*sin(q4) - cos(q4)*(cos(q1)*cos(q2)*cos(q3) + cos(q1)*sin(q2)*sin(q3))))/2000 - (37*dq4*sin(q4)*(cos(q1)*cos(q2)*cos(q3) + cos(q1)*sin(q2)*sin(q3)))/1000, (37*cos(q5)*(cos(q4)*(dq1*cos(q2)*cos(q3)*sin(q1) - dq2*cos(q1)*cos(q2)*sin(q3) + dq2*cos(q1)*cos(q3)*sin(q2) + dq3*cos(q1)*cos(q2)*sin(q3) - dq3*cos(q1)*cos(q3)*sin(q2) + dq1*sin(q1)*sin(q2)*sin(q3)) + dq1*cos(q1)*sin(q4) + dq4*cos(q4)*sin(q1) + dq4*sin(q4)*(cos(q1)*cos(q2)*cos(q3) + cos(q1)*sin(q2)*sin(q3))))/1000 - (37*sin(q5)*(sin(q4)*(dq1*cos(q2)*cos(q3)*sin(q1) - dq2*cos(q1)*cos(q2)*sin(q3) + dq2*cos(q1)*cos(q3)*sin(q2) + dq3*cos(q1)*cos(q2)*sin(q3) - dq3*cos(q1)*cos(q3)*sin(q2) + dq1*sin(q1)*sin(q2)*sin(q3)) - dq1*cos(q1)*cos(q4) + dq4*sin(q1)*sin(q4) - dq4*cos(q4)*(cos(q1)*cos(q2)*cos(q3) + cos(q1)*sin(q2)*sin(q3))))/2000 + (29*3^(1/2)*(cos(q5)*(cos(q4)*(dq1*cos(q2)*cos(q3)*sin(q1) - dq2*cos(q1)*cos(q2)*sin(q3) + dq2*cos(q1)*cos(q3)*sin(q2) + dq3*cos(q1)*cos(q2)*sin(q3) - dq3*cos(q1)*cos(q3)*sin(q2) + dq1*sin(q1)*sin(q2)*sin(q3)) + dq1*cos(q1)*sin(q4) + dq4*cos(q4)*sin(q1) + dq4*sin(q4)*(cos(q1)*cos(q2)*cos(q3) + cos(q1)*sin(q2)*sin(q3))) - (sin(q5)*(sin(q4)*(dq1*cos(q2)*cos(q3)*sin(q1) - dq2*cos(q1)*cos(q2)*sin(q3) + dq2*cos(q1)*cos(q3)*sin(q2) + dq3*cos(q1)*cos(q2)*sin(q3) - dq3*cos(q1)*cos(q3)*sin(q2) + dq1*sin(q1)*sin(q2)*sin(q3)) - dq1*cos(q1)*cos(q4) + dq4*sin(q1)*sin(q4) - dq4*cos(q4)*(cos(q1)*cos(q2)*cos(q3) + cos(q1)*sin(q2)*sin(q3))))/2 + (3^(1/2)*sin(q5)*(dq2*cos(q1)*cos(q2)*cos(q3) - dq3*cos(q1)*cos(q2)*cos(q3) + dq1*cos(q2)*sin(q1)*sin(q3) - dq1*cos(q3)*sin(q1)*sin(q2) + dq2*cos(q1)*sin(q2)*sin(q3) - dq3*cos(q1)*sin(q2)*sin(q3)))/2 + (dq5*cos(q5)*(cos(q4)*sin(q1) + sin(q4)*(cos(q1)*cos(q2)*cos(q3) + cos(q1)*sin(q2)*sin(q3))))/2 - dq5*sin(q5)*(sin(q1)*sin(q4) - cos(q4)*(cos(q1)*cos(q2)*cos(q3) + cos(q1)*sin(q2)*sin(q3))) - (3^(1/2)*dq5*cos(q5)*(cos(q1)*cos(q2)*sin(q3) - cos(q1)*cos(q3)*sin(q2)))/2))/625 + (37*3^(1/2)*sin(q5)*(dq2*cos(q1)*cos(q2)*cos(q3) - dq3*cos(q1)*cos(q2)*cos(q3) + dq1*cos(q2)*sin(q1)*sin(q3) - dq1*cos(q3)*sin(q1)*sin(q2) + dq2*cos(q1)*sin(q2)*sin(q3) - dq3*cos(q1)*sin(q2)*sin(q3)))/2000 + (37*dq5*cos(q5)*(cos(q4)*sin(q1) + sin(q4)*(cos(q1)*cos(q2)*cos(q3) + cos(q1)*sin(q2)*sin(q3))))/2000 - (37*dq5*sin(q5)*(sin(q1)*sin(q4) - cos(q4)*(cos(q1)*cos(q2)*cos(q3) + cos(q1)*sin(q2)*sin(q3))))/1000 - (37*3^(1/2)*dq5*cos(q5)*(cos(q1)*cos(q2)*sin(q3) - cos(q1)*cos(q3)*sin(q2)))/2000,                                                                                                                                                                                                                                                                                                                                                                                                                                                                                                                                                                                                                                                                                                                                                                                                                                                                                                                                                                                                                                                                                                                                                                                                                                                                                                                                                                                                                                                                                                                                                                                                                                                                                         0;
(221*3^(1/2)*(sin(q4)*(dq1*cos(q2)*cos(q3)*sin(q1) - dq2*cos(q1)*cos(q2)*sin(q3) + dq2*cos(q1)*cos(q3)*sin(q2) + dq3*cos(q1)*cos(q2)*sin(q3) - dq3*cos(q1)*cos(q3)*sin(q2) + dq1*sin(q1)*sin(q2)*sin(q3)) - dq1*cos(q1)*cos(q4) + dq4*sin(q1)*sin(q4) - dq4*cos(q4)*(cos(q1)*cos(q2)*cos(q3) + cos(q1)*sin(q2)*sin(q3))))/4000 - (37*sin(q5)*(cos(q4)*(dq1*cos(q2)*cos(q3)*sin(q1) - dq2*cos(q1)*cos(q2)*sin(q3) + dq2*cos(q1)*cos(q3)*sin(q2) + dq3*cos(q1)*cos(q2)*sin(q3) - dq3*cos(q1)*cos(q3)*sin(q2) + dq1*sin(q1)*sin(q2)*sin(q3)) + dq1*cos(q1)*sin(q4) + dq4*cos(q4)*sin(q1) + dq4*sin(q4)*(cos(q1)*cos(q2)*cos(q3) + cos(q1)*sin(q2)*sin(q3))))/1000 - (37*cos(q5)*(sin(q4)*(dq1*cos(q2)*cos(q3)*sin(q1) - dq2*cos(q1)*cos(q2)*sin(q3) + dq2*cos(q1)*cos(q3)*sin(q2) + dq3*cos(q1)*cos(q2)*sin(q3) - dq3*cos(q1)*cos(q3)*sin(q2) + dq1*sin(q1)*sin(q2)*sin(q3)) - dq1*cos(q1)*cos(q4) + dq4*sin(q1)*sin(q4) - dq4*cos(q4)*(cos(q1)*cos(q2)*cos(q3) + cos(q1)*sin(q2)*sin(q3))))/2000 + (7*dq1*cos(q1))/1000 - (29*3^(1/2)*((cos(q5)*(sin(q4)*(dq1*cos(q2)*cos(q3)*sin(q1) - dq2*cos(q1)*cos(q2)*sin(q3) + dq2*cos(q1)*cos(q3)*sin(q2) + dq3*cos(q1)*cos(q2)*sin(q3) - dq3*cos(q1)*cos(q3)*sin(q2) + dq1*sin(q1)*sin(q2)*sin(q3)) - dq1*cos(q1)*cos(q4) + dq4*sin(q1)*sin(q4) - dq4*cos(q4)*(cos(q1)*cos(q2)*cos(q3) + cos(q1)*sin(q2)*sin(q3))))/2 + sin(q5)*(cos(q4)*(dq1*cos(q2)*cos(q3)*sin(q1) - dq2*cos(q1)*cos(q2)*sin(q3) + dq2*cos(q1)*cos(q3)*sin(q2) + dq3*cos(q1)*cos(q2)*sin(q3) - dq3*cos(q1)*cos(q3)*sin(q2) + dq1*sin(q1)*sin(q2)*sin(q3)) + dq1*cos(q1)*sin(q4) + dq4*cos(q4)*sin(q1) + dq4*sin(q4)*(cos(q1)*cos(q2)*cos(q3) + cos(q1)*sin(q2)*sin(q3))) + dq5*cos(q5)*(sin(q1)*sin(q4) - cos(q4)*(cos(q1)*cos(q2)*cos(q3) + cos(q1)*sin(q2)*sin(q3))) + (dq5*sin(q5)*(cos(q4)*sin(q1) + sin(q4)*(cos(q1)*cos(q2)*cos(q3) + cos(q1)*sin(q2)*sin(q3))))/2 - (3^(1/2)*cos(q5)*(dq2*cos(q1)*cos(q2)*cos(q3) - dq3*cos(q1)*cos(q2)*cos(q3) + dq1*cos(q2)*sin(q1)*sin(q3) - dq1*cos(q3)*sin(q1)*sin(q2) + dq2*cos(q1)*sin(q2)*sin(q3) - dq3*cos(q1)*sin(q2)*sin(q3)))/2 - (3^(1/2)*dq5*sin(q5)*(cos(q1)*cos(q2)*sin(q3) - cos(q1)*cos(q3)*sin(q2)))/2))/625 + (37*sin(q4)*(dq1*cos(q2)*cos(q3)*sin(q1) - dq2*cos(q1)*cos(q2)*sin(q3) + dq2*cos(q1)*cos(q3)*sin(q2) + dq3*cos(q1)*cos(q2)*sin(q3) - dq3*cos(q1)*cos(q3)*sin(q2) + dq1*sin(q1)*sin(q2)*sin(q3)))/1000 - (29*dq2*cos(q1)*cos(q2))/100 - (37*dq1*cos(q1)*cos(q4))/1000 + (29*dq1*sin(q1)*sin(q2))/100 + (37*dq4*sin(q1)*sin(q4))/1000 - (37*dq5*cos(q5)*(sin(q1)*sin(q4) - cos(q4)*(cos(q1)*cos(q2)*cos(q3) + cos(q1)*sin(q2)*sin(q3))))/1000 - (37*dq5*sin(q5)*(cos(q4)*sin(q1) + sin(q4)*(cos(q1)*cos(q2)*cos(q3) + cos(q1)*sin(q2)*sin(q3))))/2000 - (37*dq4*cos(q4)*(cos(q1)*cos(q2)*cos(q3) + cos(q1)*sin(q2)*sin(q3)))/1000 + (37*3^(1/2)*cos(q5)*(dq2*cos(q1)*cos(q2)*cos(q3) - dq3*cos(q1)*cos(q2)*cos(q3) + dq1*cos(q2)*sin(q1)*sin(q3) - dq1*cos(q3)*sin(q1)*sin(q2) + dq2*cos(q1)*sin(q2)*sin(q3) - dq3*cos(q1)*sin(q2)*sin(q3)))/2000 + (37*3^(1/2)*dq5*sin(q5)*(cos(q1)*cos(q2)*sin(q3) - cos(q1)*cos(q3)*sin(q2)))/2000 + (4849*dq2*cos(q1)*cos(q2)*cos(q3))/20000 - (4849*dq3*cos(q1)*cos(q2)*cos(q3))/20000 + (4849*dq1*cos(q2)*sin(q1)*sin(q3))/20000 - (4849*dq1*cos(q3)*sin(q1)*sin(q2))/20000 + (4849*dq2*cos(q1)*sin(q2)*sin(q3))/20000 - (4849*dq3*cos(q1)*sin(q2)*sin(q3))/20000, (29*3^(1/2)*((3^(1/2)*cos(q5)*(dq1*cos(q1)*cos(q2)*cos(q3) + dq1*cos(q1)*sin(q2)*sin(q3) + dq2*cos(q2)*sin(q1)*sin(q3) - dq2*cos(q3)*sin(q1)*sin(q2) - dq3*cos(q2)*sin(q1)*sin(q3) + dq3*cos(q3)*sin(q1)*sin(q2)))/2 + cos(q4)*sin(q5)*(dq1*cos(q1)*cos(q2)*sin(q3) - dq1*cos(q1)*cos(q3)*sin(q2) - dq2*cos(q2)*cos(q3)*sin(q1) + dq3*cos(q2)*cos(q3)*sin(q1) - dq2*sin(q1)*sin(q2)*sin(q3) + dq3*sin(q1)*sin(q2)*sin(q3)) + (cos(q5)*sin(q4)*(dq1*cos(q1)*cos(q2)*sin(q3) - dq1*cos(q1)*cos(q3)*sin(q2) - dq2*cos(q2)*cos(q3)*sin(q1) + dq3*cos(q2)*cos(q3)*sin(q1) - dq2*sin(q1)*sin(q2)*sin(q3) + dq3*sin(q1)*sin(q2)*sin(q3)))/2 - (3^(1/2)*dq5*sin(q5)*(sin(q1)*sin(q2)*sin(q3) + cos(q2)*cos(q3)*sin(q1)))/2 + (dq4*cos(q4)*cos(q5)*(cos(q2)*sin(q1)*sin(q3) - cos(q3)*sin(q1)*sin(q2)))/2 + dq5*cos(q4)*cos(q5)*(cos(q2)*sin(q1)*sin(q3) - cos(q3)*sin(q1)*sin(q2)) - dq4*sin(q4)*sin(q5)*(cos(q2)*sin(q1)*sin(q3) - cos(q3)*sin(q1)*sin(q2)) - (dq5*sin(q4)*sin(q5)*(cos(q2)*sin(q1)*sin(q3) - cos(q3)*sin(q1)*sin(q2)))/2))/625 - (37*sin(q4)*(dq1*cos(q1)*cos(q2)*sin(q3) - dq1*cos(q1)*cos(q3)*sin(q2) - dq2*cos(q2)*cos(q3)*sin(q1) + dq3*cos(q2)*cos(q3)*sin(q1) - dq2*sin(q1)*sin(q2)*sin(q3) + dq3*sin(q1)*sin(q2)*sin(q3)))/1000 + (37*3^(1/2)*cos(q5)*(dq1*cos(q1)*cos(q2)*cos(q3) + dq1*cos(q1)*sin(q2)*sin(q3) + dq2*cos(q2)*sin(q1)*sin(q3) - dq2*cos(q3)*sin(q1)*sin(q2) - dq3*cos(q2)*sin(q1)*sin(q3) + dq3*cos(q3)*sin(q1)*sin(q2)))/2000 - (221*3^(1/2)*sin(q4)*(dq1*cos(q1)*cos(q2)*sin(q3) - dq1*cos(q1)*cos(q3)*sin(q2) - dq2*cos(q2)*cos(q3)*sin(q1) + dq3*cos(q2)*cos(q3)*sin(q1) - dq2*sin(q1)*sin(q2)*sin(q3) + dq3*sin(q1)*sin(q2)*sin(q3)))/4000 - (29*dq1*cos(q1)*cos(q2))/100 + (29*dq2*sin(q1)*sin(q2))/100 + (37*cos(q4)*sin(q5)*(dq1*cos(q1)*cos(q2)*sin(q3) - dq1*cos(q1)*cos(q3)*sin(q2) - dq2*cos(q2)*cos(q3)*sin(q1) + dq3*cos(q2)*cos(q3)*sin(q1) - dq2*sin(q1)*sin(q2)*sin(q3) + dq3*sin(q1)*sin(q2)*sin(q3)))/1000 + (37*cos(q5)*sin(q4)*(dq1*cos(q1)*cos(q2)*sin(q3) - dq1*cos(q1)*cos(q3)*sin(q2) - dq2*cos(q2)*cos(q3)*sin(q1) + dq3*cos(q2)*cos(q3)*sin(q1) - dq2*sin(q1)*sin(q2)*sin(q3) + dq3*sin(q1)*sin(q2)*sin(q3)))/2000 - (37*dq4*cos(q4)*(cos(q2)*sin(q1)*sin(q3) - cos(q3)*sin(q1)*sin(q2)))/1000 + (4849*dq1*cos(q1)*cos(q2)*cos(q3))/20000 - (221*3^(1/2)*dq4*cos(q4)*(cos(q2)*sin(q1)*sin(q3) - cos(q3)*sin(q1)*sin(q2)))/4000 - (37*3^(1/2)*dq5*sin(q5)*(sin(q1)*sin(q2)*sin(q3) + cos(q2)*cos(q3)*sin(q1)))/2000 + (4849*dq1*cos(q1)*sin(q2)*sin(q3))/20000 + (4849*dq2*cos(q2)*sin(q1)*sin(q3))/20000 - (4849*dq2*cos(q3)*sin(q1)*sin(q2))/20000 - (4849*dq3*cos(q2)*sin(q1)*sin(q3))/20000 + (4849*dq3*cos(q3)*sin(q1)*sin(q2))/20000 + (37*dq4*cos(q4)*cos(q5)*(cos(q2)*sin(q1)*sin(q3) - cos(q3)*sin(q1)*sin(q2)))/2000 + (37*dq5*cos(q4)*cos(q5)*(cos(q2)*sin(q1)*sin(q3) - cos(q3)*sin(q1)*sin(q2)))/1000 - (37*dq4*sin(q4)*sin(q5)*(cos(q2)*sin(q1)*sin(q3) - cos(q3)*sin(q1)*sin(q2)))/1000 - (37*dq5*sin(q4)*sin(q5)*(cos(q2)*sin(q1)*sin(q3) - cos(q3)*sin(q1)*sin(q2)))/2000, (37*sin(q4)*(dq1*cos(q1)*cos(q2)*sin(q3) - dq1*cos(q1)*cos(q3)*sin(q2) - dq2*cos(q2)*cos(q3)*sin(q1) + dq3*cos(q2)*cos(q3)*sin(q1) - dq2*sin(q1)*sin(q2)*sin(q3) + dq3*sin(q1)*sin(q2)*sin(q3)))/1000 - (29*3^(1/2)*((3^(1/2)*cos(q5)*(dq1*cos(q1)*cos(q2)*cos(q3) + dq1*cos(q1)*sin(q2)*sin(q3) + dq2*cos(q2)*sin(q1)*sin(q3) - dq2*cos(q3)*sin(q1)*sin(q2) - dq3*cos(q2)*sin(q1)*sin(q3) + dq3*cos(q3)*sin(q1)*sin(q2)))/2 + cos(q4)*sin(q5)*(dq1*cos(q1)*cos(q2)*sin(q3) - dq1*cos(q1)*cos(q3)*sin(q2) - dq2*cos(q2)*cos(q3)*sin(q1) + dq3*cos(q2)*cos(q3)*sin(q1) - dq2*sin(q1)*sin(q2)*sin(q3) + dq3*sin(q1)*sin(q2)*sin(q3)) + (cos(q5)*sin(q4)*(dq1*cos(q1)*cos(q2)*sin(q3) - dq1*cos(q1)*cos(q3)*sin(q2) - dq2*cos(q2)*cos(q3)*sin(q1) + dq3*cos(q2)*cos(q3)*sin(q1) - dq2*sin(q1)*sin(q2)*sin(q3) + dq3*sin(q1)*sin(q2)*sin(q3)))/2 - (3^(1/2)*dq5*sin(q5)*(sin(q1)*sin(q2)*sin(q3) + cos(q2)*cos(q3)*sin(q1)))/2 + (dq4*cos(q4)*cos(q5)*(cos(q2)*sin(q1)*sin(q3) - cos(q3)*sin(q1)*sin(q2)))/2 + dq5*cos(q4)*cos(q5)*(cos(q2)*sin(q1)*sin(q3) - cos(q3)*sin(q1)*sin(q2)) - dq4*sin(q4)*sin(q5)*(cos(q2)*sin(q1)*sin(q3) - cos(q3)*sin(q1)*sin(q2)) - (dq5*sin(q4)*sin(q5)*(cos(q2)*sin(q1)*sin(q3) - cos(q3)*sin(q1)*sin(q2)))/2))/625 - (37*3^(1/2)*cos(q5)*(dq1*cos(q1)*cos(q2)*cos(q3) + dq1*cos(q1)*sin(q2)*sin(q3) + dq2*cos(q2)*sin(q1)*sin(q3) - dq2*cos(q3)*sin(q1)*sin(q2) - dq3*cos(q2)*sin(q1)*sin(q3) + dq3*cos(q3)*sin(q1)*sin(q2)))/2000 + (221*3^(1/2)*sin(q4)*(dq1*cos(q1)*cos(q2)*sin(q3) - dq1*cos(q1)*cos(q3)*sin(q2) - dq2*cos(q2)*cos(q3)*sin(q1) + dq3*cos(q2)*cos(q3)*sin(q1) - dq2*sin(q1)*sin(q2)*sin(q3) + dq3*sin(q1)*sin(q2)*sin(q3)))/4000 - (37*cos(q4)*sin(q5)*(dq1*cos(q1)*cos(q2)*sin(q3) - dq1*cos(q1)*cos(q3)*sin(q2) - dq2*cos(q2)*cos(q3)*sin(q1) + dq3*cos(q2)*cos(q3)*sin(q1) - dq2*sin(q1)*sin(q2)*sin(q3) + dq3*sin(q1)*sin(q2)*sin(q3)))/1000 - (37*cos(q5)*sin(q4)*(dq1*cos(q1)*cos(q2)*sin(q3) - dq1*cos(q1)*cos(q3)*sin(q2) - dq2*cos(q2)*cos(q3)*sin(q1) + dq3*cos(q2)*cos(q3)*sin(q1) - dq2*sin(q1)*sin(q2)*sin(q3) + dq3*sin(q1)*sin(q2)*sin(q3)))/2000 + (37*dq4*cos(q4)*(cos(q2)*sin(q1)*sin(q3) - cos(q3)*sin(q1)*sin(q2)))/1000 - (4849*dq1*cos(q1)*cos(q2)*cos(q3))/20000 + (221*3^(1/2)*dq4*cos(q4)*(cos(q2)*sin(q1)*sin(q3) - cos(q3)*sin(q1)*sin(q2)))/4000 + (37*3^(1/2)*dq5*sin(q5)*(sin(q1)*sin(q2)*sin(q3) + cos(q2)*cos(q3)*sin(q1)))/2000 - (4849*dq1*cos(q1)*sin(q2)*sin(q3))/20000 - (4849*dq2*cos(q2)*sin(q1)*sin(q3))/20000 + (4849*dq2*cos(q3)*sin(q1)*sin(q2))/20000 + (4849*dq3*cos(q2)*sin(q1)*sin(q3))/20000 - (4849*dq3*cos(q3)*sin(q1)*sin(q2))/20000 - (37*dq4*cos(q4)*cos(q5)*(cos(q2)*sin(q1)*sin(q3) - cos(q3)*sin(q1)*sin(q2)))/2000 - (37*dq5*cos(q4)*cos(q5)*(cos(q2)*sin(q1)*sin(q3) - cos(q3)*sin(q1)*sin(q2)))/1000 + (37*dq4*sin(q4)*sin(q5)*(cos(q2)*sin(q1)*sin(q3) - cos(q3)*sin(q1)*sin(q2)))/1000 + (37*dq5*sin(q4)*sin(q5)*(cos(q2)*sin(q1)*sin(q3) - cos(q3)*sin(q1)*sin(q2)))/2000, (29*3^(1/2)*((cos(q5)*(cos(q4)*(dq1*cos(q1)*cos(q2)*cos(q3) + dq1*cos(q1)*sin(q2)*sin(q3) + dq2*cos(q2)*sin(q1)*sin(q3) - dq2*cos(q3)*sin(q1)*sin(q2) - dq3*cos(q2)*sin(q1)*sin(q3) + dq3*cos(q3)*sin(q1)*sin(q2)) - dq4*sin(q4)*(sin(q1)*sin(q2)*sin(q3) + cos(q2)*cos(q3)*sin(q1)) + dq4*cos(q1)*cos(q4) - dq1*sin(q1)*sin(q4)))/2 - sin(q5)*(sin(q4)*(dq1*cos(q1)*cos(q2)*cos(q3) + dq1*cos(q1)*sin(q2)*sin(q3) + dq2*cos(q2)*sin(q1)*sin(q3) - dq2*cos(q3)*sin(q1)*sin(q2) - dq3*cos(q2)*sin(q1)*sin(q3) + dq3*cos(q3)*sin(q1)*sin(q2)) + dq1*cos(q4)*sin(q1) + dq4*cos(q1)*sin(q4) + dq4*cos(q4)*(sin(q1)*sin(q2)*sin(q3) + cos(q2)*cos(q3)*sin(q1))) + dq5*cos(q5)*(cos(q1)*cos(q4) - sin(q4)*(sin(q1)*sin(q2)*sin(q3) + cos(q2)*cos(q3)*sin(q1))) - (dq5*sin(q5)*(cos(q1)*sin(q4) + cos(q4)*(sin(q1)*sin(q2)*sin(q3) + cos(q2)*cos(q3)*sin(q1))))/2))/625 + (37*cos(q5)*(cos(q4)*(dq1*cos(q1)*cos(q2)*cos(q3) + dq1*cos(q1)*sin(q2)*sin(q3) + dq2*cos(q2)*sin(q1)*sin(q3) - dq2*cos(q3)*sin(q1)*sin(q2) - dq3*cos(q2)*sin(q1)*sin(q3) + dq3*cos(q3)*sin(q1)*sin(q2)) - dq4*sin(q4)*(sin(q1)*sin(q2)*sin(q3) + cos(q2)*cos(q3)*sin(q1)) + dq4*cos(q1)*cos(q4) - dq1*sin(q1)*sin(q4)))/2000 - (37*sin(q5)*(sin(q4)*(dq1*cos(q1)*cos(q2)*cos(q3) + dq1*cos(q1)*sin(q2)*sin(q3) + dq2*cos(q2)*sin(q1)*sin(q3) - dq2*cos(q3)*sin(q1)*sin(q2) - dq3*cos(q2)*sin(q1)*sin(q3) + dq3*cos(q3)*sin(q1)*sin(q2)) + dq1*cos(q4)*sin(q1) + dq4*cos(q1)*sin(q4) + dq4*cos(q4)*(sin(q1)*sin(q2)*sin(q3) + cos(q2)*cos(q3)*sin(q1))))/1000 - (37*cos(q4)*(dq1*cos(q1)*cos(q2)*cos(q3) + dq1*cos(q1)*sin(q2)*sin(q3) + dq2*cos(q2)*sin(q1)*sin(q3) - dq2*cos(q3)*sin(q1)*sin(q2) - dq3*cos(q2)*sin(q1)*sin(q3) + dq3*cos(q3)*sin(q1)*sin(q2)))/1000 - (221*3^(1/2)*(cos(q4)*(dq1*cos(q1)*cos(q2)*cos(q3) + dq1*cos(q1)*sin(q2)*sin(q3) + dq2*cos(q2)*sin(q1)*sin(q3) - dq2*cos(q3)*sin(q1)*sin(q2) - dq3*cos(q2)*sin(q1)*sin(q3) + dq3*cos(q3)*sin(q1)*sin(q2)) - dq4*sin(q4)*(sin(q1)*sin(q2)*sin(q3) + cos(q2)*cos(q3)*sin(q1)) + dq4*cos(q1)*cos(q4) - dq1*sin(q1)*sin(q4)))/4000 + (37*dq4*sin(q4)*(sin(q1)*sin(q2)*sin(q3) + cos(q2)*cos(q3)*sin(q1)))/1000 - (37*dq4*cos(q1)*cos(q4))/1000 + (37*dq1*sin(q1)*sin(q4))/1000 + (37*dq5*cos(q5)*(cos(q1)*cos(q4) - sin(q4)*(sin(q1)*sin(q2)*sin(q3) + cos(q2)*cos(q3)*sin(q1))))/1000 - (37*dq5*sin(q5)*(cos(q1)*sin(q4) + cos(q4)*(sin(q1)*sin(q2)*sin(q3) + cos(q2)*cos(q3)*sin(q1))))/2000, (37*cos(q5)*(cos(q4)*(dq1*cos(q1)*cos(q2)*cos(q3) + dq1*cos(q1)*sin(q2)*sin(q3) + dq2*cos(q2)*sin(q1)*sin(q3) - dq2*cos(q3)*sin(q1)*sin(q2) - dq3*cos(q2)*sin(q1)*sin(q3) + dq3*cos(q3)*sin(q1)*sin(q2)) - dq4*sin(q4)*(sin(q1)*sin(q2)*sin(q3) + cos(q2)*cos(q3)*sin(q1)) + dq4*cos(q1)*cos(q4) - dq1*sin(q1)*sin(q4)))/1000 - (37*sin(q5)*(sin(q4)*(dq1*cos(q1)*cos(q2)*cos(q3) + dq1*cos(q1)*sin(q2)*sin(q3) + dq2*cos(q2)*sin(q1)*sin(q3) - dq2*cos(q3)*sin(q1)*sin(q2) - dq3*cos(q2)*sin(q1)*sin(q3) + dq3*cos(q3)*sin(q1)*sin(q2)) + dq1*cos(q4)*sin(q1) + dq4*cos(q1)*sin(q4) + dq4*cos(q4)*(sin(q1)*sin(q2)*sin(q3) + cos(q2)*cos(q3)*sin(q1))))/2000 + (29*3^(1/2)*(cos(q5)*(cos(q4)*(dq1*cos(q1)*cos(q2)*cos(q3) + dq1*cos(q1)*sin(q2)*sin(q3) + dq2*cos(q2)*sin(q1)*sin(q3) - dq2*cos(q3)*sin(q1)*sin(q2) - dq3*cos(q2)*sin(q1)*sin(q3) + dq3*cos(q3)*sin(q1)*sin(q2)) - dq4*sin(q4)*(sin(q1)*sin(q2)*sin(q3) + cos(q2)*cos(q3)*sin(q1)) + dq4*cos(q1)*cos(q4) - dq1*sin(q1)*sin(q4)) - (sin(q5)*(sin(q4)*(dq1*cos(q1)*cos(q2)*cos(q3) + dq1*cos(q1)*sin(q2)*sin(q3) + dq2*cos(q2)*sin(q1)*sin(q3) - dq2*cos(q3)*sin(q1)*sin(q2) - dq3*cos(q2)*sin(q1)*sin(q3) + dq3*cos(q3)*sin(q1)*sin(q2)) + dq1*cos(q4)*sin(q1) + dq4*cos(q1)*sin(q4) + dq4*cos(q4)*(sin(q1)*sin(q2)*sin(q3) + cos(q2)*cos(q3)*sin(q1))))/2 + (3^(1/2)*sin(q5)*(dq1*cos(q1)*cos(q2)*sin(q3) - dq1*cos(q1)*cos(q3)*sin(q2) - dq2*cos(q2)*cos(q3)*sin(q1) + dq3*cos(q2)*cos(q3)*sin(q1) - dq2*sin(q1)*sin(q2)*sin(q3) + dq3*sin(q1)*sin(q2)*sin(q3)))/2 + (dq5*cos(q5)*(cos(q1)*cos(q4) - sin(q4)*(sin(q1)*sin(q2)*sin(q3) + cos(q2)*cos(q3)*sin(q1))))/2 - dq5*sin(q5)*(cos(q1)*sin(q4) + cos(q4)*(sin(q1)*sin(q2)*sin(q3) + cos(q2)*cos(q3)*sin(q1))) + (3^(1/2)*dq5*cos(q5)*(cos(q2)*sin(q1)*sin(q3) - cos(q3)*sin(q1)*sin(q2)))/2))/625 + (37*3^(1/2)*sin(q5)*(dq1*cos(q1)*cos(q2)*sin(q3) - dq1*cos(q1)*cos(q3)*sin(q2) - dq2*cos(q2)*cos(q3)*sin(q1) + dq3*cos(q2)*cos(q3)*sin(q1) - dq2*sin(q1)*sin(q2)*sin(q3) + dq3*sin(q1)*sin(q2)*sin(q3)))/2000 + (37*dq5*cos(q5)*(cos(q1)*cos(q4) - sin(q4)*(sin(q1)*sin(q2)*sin(q3) + cos(q2)*cos(q3)*sin(q1))))/2000 - (37*dq5*sin(q5)*(cos(q1)*sin(q4) + cos(q4)*(sin(q1)*sin(q2)*sin(q3) + cos(q2)*cos(q3)*sin(q1))))/1000 + (37*3^(1/2)*dq5*cos(q5)*(cos(q2)*sin(q1)*sin(q3) - cos(q3)*sin(q1)*sin(q2)))/2000,                                                                                                                                                                                                                                                                                                                                                                                                                                                                                                                                                                                                                                                                                                                                                                                                                                                                                                                                                                                                                                                                                                                                                                                                                                                                                                                                                                                                                                                                                                                                                                                                                                                                                         0;
                                                                                                                                                                                                                                                                                                                                                                                                                                                                                                                                                                                                                                                                                                                                                                                                                                                                                                                                                                                                                                                                                                                                                                                                                                                                                                                                                                                                                                                                                                                                                                                                                                                                                                                                                                                                                                                                                                                                                                                                                                                                                                                                                                                                                                                                                                                                                                                                                                                                                                                                                                                                                                                                                                                                                                                                                                                                                                                                                                                                                                                                                                                                                                                                                                                                                                                                                                                       0,                                                                                                                                                                                                                                                                                                                                                                                                                                                                                                                                                                                                                                                                                                                                                                                                                                                                                                                                                                                                                                                                                                                              (37*sin(q4)*(dq2*cos(q2)*sin(q3) - dq2*cos(q3)*sin(q2) - dq3*cos(q2)*sin(q3) + dq3*cos(q3)*sin(q2)))/1000 + (29*dq2*cos(q2))/100 - (29*3^(1/2)*(cos(q4)*sin(q5)*(dq2*cos(q2)*sin(q3) - dq2*cos(q3)*sin(q2) - dq3*cos(q2)*sin(q3) + dq3*cos(q3)*sin(q2)) + (cos(q5)*sin(q4)*(dq2*cos(q2)*sin(q3) - dq2*cos(q3)*sin(q2) - dq3*cos(q2)*sin(q3) + dq3*cos(q3)*sin(q2)))/2 + (3^(1/2)*cos(q5)*(dq2*cos(q2)*cos(q3) - dq3*cos(q2)*cos(q3) + dq2*sin(q2)*sin(q3) - dq3*sin(q2)*sin(q3)))/2 - dq4*sin(q4)*sin(q5)*(cos(q2)*cos(q3) + sin(q2)*sin(q3)) - (dq5*sin(q4)*sin(q5)*(cos(q2)*cos(q3) + sin(q2)*sin(q3)))/2 + (3^(1/2)*dq5*sin(q5)*(cos(q2)*sin(q3) - cos(q3)*sin(q2)))/2 + (dq4*cos(q4)*cos(q5)*(cos(q2)*cos(q3) + sin(q2)*sin(q3)))/2 + dq5*cos(q4)*cos(q5)*(cos(q2)*cos(q3) + sin(q2)*sin(q3))))/625 + (37*dq4*cos(q4)*(cos(q2)*cos(q3) + sin(q2)*sin(q3)))/1000 - (37*cos(q4)*sin(q5)*(dq2*cos(q2)*sin(q3) - dq2*cos(q3)*sin(q2) - dq3*cos(q2)*sin(q3) + dq3*cos(q3)*sin(q2)))/1000 - (37*cos(q5)*sin(q4)*(dq2*cos(q2)*sin(q3) - dq2*cos(q3)*sin(q2) - dq3*cos(q2)*sin(q3) + dq3*cos(q3)*sin(q2)))/2000 - (4849*dq2*cos(q2)*cos(q3))/20000 + (4849*dq3*cos(q2)*cos(q3))/20000 - (4849*dq2*sin(q2)*sin(q3))/20000 + (4849*dq3*sin(q2)*sin(q3))/20000 - (37*3^(1/2)*cos(q5)*(dq2*cos(q2)*cos(q3) - dq3*cos(q2)*cos(q3) + dq2*sin(q2)*sin(q3) - dq3*sin(q2)*sin(q3)))/2000 + (221*3^(1/2)*sin(q4)*(dq2*cos(q2)*sin(q3) - dq2*cos(q3)*sin(q2) - dq3*cos(q2)*sin(q3) + dq3*cos(q3)*sin(q2)))/4000 + (37*dq4*sin(q4)*sin(q5)*(cos(q2)*cos(q3) + sin(q2)*sin(q3)))/1000 + (37*dq5*sin(q4)*sin(q5)*(cos(q2)*cos(q3) + sin(q2)*sin(q3)))/2000 + (221*3^(1/2)*dq4*cos(q4)*(cos(q2)*cos(q3) + sin(q2)*sin(q3)))/4000 - (37*3^(1/2)*dq5*sin(q5)*(cos(q2)*sin(q3) - cos(q3)*sin(q2)))/2000 - (37*dq4*cos(q4)*cos(q5)*(cos(q2)*cos(q3) + sin(q2)*sin(q3)))/2000 - (37*dq5*cos(q4)*cos(q5)*(cos(q2)*cos(q3) + sin(q2)*sin(q3)))/1000,                                                                                                                                                                                                                                                                                                                                                                                                                                                                                                                                                                                                                                                                                                                                                                                                                                                                                                                                                                                                                                                                                       (29*3^(1/2)*(cos(q4)*sin(q5)*(dq2*cos(q2)*sin(q3) - dq2*cos(q3)*sin(q2) - dq3*cos(q2)*sin(q3) + dq3*cos(q3)*sin(q2)) + (cos(q5)*sin(q4)*(dq2*cos(q2)*sin(q3) - dq2*cos(q3)*sin(q2) - dq3*cos(q2)*sin(q3) + dq3*cos(q3)*sin(q2)))/2 + (3^(1/2)*cos(q5)*(dq2*cos(q2)*cos(q3) - dq3*cos(q2)*cos(q3) + dq2*sin(q2)*sin(q3) - dq3*sin(q2)*sin(q3)))/2 - dq4*sin(q4)*sin(q5)*(cos(q2)*cos(q3) + sin(q2)*sin(q3)) - (dq5*sin(q4)*sin(q5)*(cos(q2)*cos(q3) + sin(q2)*sin(q3)))/2 + (3^(1/2)*dq5*sin(q5)*(cos(q2)*sin(q3) - cos(q3)*sin(q2)))/2 + (dq4*cos(q4)*cos(q5)*(cos(q2)*cos(q3) + sin(q2)*sin(q3)))/2 + dq5*cos(q4)*cos(q5)*(cos(q2)*cos(q3) + sin(q2)*sin(q3))))/625 - (37*sin(q4)*(dq2*cos(q2)*sin(q3) - dq2*cos(q3)*sin(q2) - dq3*cos(q2)*sin(q3) + dq3*cos(q3)*sin(q2)))/1000 - (37*dq4*cos(q4)*(cos(q2)*cos(q3) + sin(q2)*sin(q3)))/1000 + (37*cos(q4)*sin(q5)*(dq2*cos(q2)*sin(q3) - dq2*cos(q3)*sin(q2) - dq3*cos(q2)*sin(q3) + dq3*cos(q3)*sin(q2)))/1000 + (37*cos(q5)*sin(q4)*(dq2*cos(q2)*sin(q3) - dq2*cos(q3)*sin(q2) - dq3*cos(q2)*sin(q3) + dq3*cos(q3)*sin(q2)))/2000 + (4849*dq2*cos(q2)*cos(q3))/20000 - (4849*dq3*cos(q2)*cos(q3))/20000 + (4849*dq2*sin(q2)*sin(q3))/20000 - (4849*dq3*sin(q2)*sin(q3))/20000 + (37*3^(1/2)*cos(q5)*(dq2*cos(q2)*cos(q3) - dq3*cos(q2)*cos(q3) + dq2*sin(q2)*sin(q3) - dq3*sin(q2)*sin(q3)))/2000 - (221*3^(1/2)*sin(q4)*(dq2*cos(q2)*sin(q3) - dq2*cos(q3)*sin(q2) - dq3*cos(q2)*sin(q3) + dq3*cos(q3)*sin(q2)))/4000 - (37*dq4*sin(q4)*sin(q5)*(cos(q2)*cos(q3) + sin(q2)*sin(q3)))/1000 - (37*dq5*sin(q4)*sin(q5)*(cos(q2)*cos(q3) + sin(q2)*sin(q3)))/2000 - (221*3^(1/2)*dq4*cos(q4)*(cos(q2)*cos(q3) + sin(q2)*sin(q3)))/4000 + (37*3^(1/2)*dq5*sin(q5)*(cos(q2)*sin(q3) - cos(q3)*sin(q2)))/2000 + (37*dq4*cos(q4)*cos(q5)*(cos(q2)*cos(q3) + sin(q2)*sin(q3)))/2000 + (37*dq5*cos(q4)*cos(q5)*(cos(q2)*cos(q3) + sin(q2)*sin(q3)))/1000,                                                                                                                                                                                                                                                                                                                                                                                                                                                                                                                                                                                                                                                                                                                                                                                                                                                                                                                                                                                                                                                    (37*cos(q4)*(dq2*cos(q2)*cos(q3) - dq3*cos(q2)*cos(q3) + dq2*sin(q2)*sin(q3) - dq3*sin(q2)*sin(q3)))/1000 - (29*3^(1/2)*((cos(q4)*cos(q5)*(dq2*cos(q2)*cos(q3) - dq3*cos(q2)*cos(q3) + dq2*sin(q2)*sin(q3) - dq3*sin(q2)*sin(q3)))/2 - sin(q4)*sin(q5)*(dq2*cos(q2)*cos(q3) - dq3*cos(q2)*cos(q3) + dq2*sin(q2)*sin(q3) - dq3*sin(q2)*sin(q3)) + dq4*cos(q4)*sin(q5)*(cos(q2)*sin(q3) - cos(q3)*sin(q2)) + (dq4*cos(q5)*sin(q4)*(cos(q2)*sin(q3) - cos(q3)*sin(q2)))/2 + (dq5*cos(q4)*sin(q5)*(cos(q2)*sin(q3) - cos(q3)*sin(q2)))/2 + dq5*cos(q5)*sin(q4)*(cos(q2)*sin(q3) - cos(q3)*sin(q2))))/625 + (37*dq4*sin(q4)*(cos(q2)*sin(q3) - cos(q3)*sin(q2)))/1000 - (37*cos(q4)*cos(q5)*(dq2*cos(q2)*cos(q3) - dq3*cos(q2)*cos(q3) + dq2*sin(q2)*sin(q3) - dq3*sin(q2)*sin(q3)))/2000 + (37*sin(q4)*sin(q5)*(dq2*cos(q2)*cos(q3) - dq3*cos(q2)*cos(q3) + dq2*sin(q2)*sin(q3) - dq3*sin(q2)*sin(q3)))/1000 + (221*3^(1/2)*cos(q4)*(dq2*cos(q2)*cos(q3) - dq3*cos(q2)*cos(q3) + dq2*sin(q2)*sin(q3) - dq3*sin(q2)*sin(q3)))/4000 - (37*dq4*cos(q4)*sin(q5)*(cos(q2)*sin(q3) - cos(q3)*sin(q2)))/1000 - (37*dq4*cos(q5)*sin(q4)*(cos(q2)*sin(q3) - cos(q3)*sin(q2)))/2000 - (37*dq5*cos(q4)*sin(q5)*(cos(q2)*sin(q3) - cos(q3)*sin(q2)))/2000 - (37*dq5*cos(q5)*sin(q4)*(cos(q2)*sin(q3) - cos(q3)*sin(q2)))/1000 + (221*3^(1/2)*dq4*sin(q4)*(cos(q2)*sin(q3) - cos(q3)*sin(q2)))/4000,                                                                                                                                                                                                                                                                                                                                                                                                                                                                                                                                                                                                                                                                                                                                                                                                                                                                                                                                                         (37*sin(q4)*sin(q5)*(dq2*cos(q2)*cos(q3) - dq3*cos(q2)*cos(q3) + dq2*sin(q2)*sin(q3) - dq3*sin(q2)*sin(q3)))/2000 - (37*cos(q4)*cos(q5)*(dq2*cos(q2)*cos(q3) - dq3*cos(q2)*cos(q3) + dq2*sin(q2)*sin(q3) - dq3*sin(q2)*sin(q3)))/1000 - (29*3^(1/2)*(cos(q4)*cos(q5)*(dq2*cos(q2)*cos(q3) - dq3*cos(q2)*cos(q3) + dq2*sin(q2)*sin(q3) - dq3*sin(q2)*sin(q3)) - (sin(q4)*sin(q5)*(dq2*cos(q2)*cos(q3) - dq3*cos(q2)*cos(q3) + dq2*sin(q2)*sin(q3) - dq3*sin(q2)*sin(q3)))/2 + (3^(1/2)*sin(q5)*(dq2*cos(q2)*sin(q3) - dq2*cos(q3)*sin(q2) - dq3*cos(q2)*sin(q3) + dq3*cos(q3)*sin(q2)))/2 + (dq4*cos(q4)*sin(q5)*(cos(q2)*sin(q3) - cos(q3)*sin(q2)))/2 + dq4*cos(q5)*sin(q4)*(cos(q2)*sin(q3) - cos(q3)*sin(q2)) + dq5*cos(q4)*sin(q5)*(cos(q2)*sin(q3) - cos(q3)*sin(q2)) + (dq5*cos(q5)*sin(q4)*(cos(q2)*sin(q3) - cos(q3)*sin(q2)))/2 + (3^(1/2)*dq5*cos(q5)*(cos(q2)*cos(q3) + sin(q2)*sin(q3)))/2))/625 - (37*3^(1/2)*sin(q5)*(dq2*cos(q2)*sin(q3) - dq2*cos(q3)*sin(q2) - dq3*cos(q2)*sin(q3) + dq3*cos(q3)*sin(q2)))/2000 - (37*dq4*cos(q4)*sin(q5)*(cos(q2)*sin(q3) - cos(q3)*sin(q2)))/2000 - (37*dq4*cos(q5)*sin(q4)*(cos(q2)*sin(q3) - cos(q3)*sin(q2)))/1000 - (37*dq5*cos(q4)*sin(q5)*(cos(q2)*sin(q3) - cos(q3)*sin(q2)))/1000 - (37*dq5*cos(q5)*sin(q4)*(cos(q2)*sin(q3) - cos(q3)*sin(q2)))/2000 - (37*3^(1/2)*dq5*cos(q5)*(cos(q2)*cos(q3) + sin(q2)*sin(q3)))/2000,                                                                                                                                                                                                                                                                                                                                                                                                                                                                                                                                                                                                                                                                                                                                                                                                                                                                                                                                                                                                                                                                                                                                                                                                                                                                                                                                                                                                                                                                                                                                                                                                                                                                                         0;
                                                                                                                                                                                                                                                                                                                                                                                                                                                                                                                                                                                                                                                                                                                                                                                                                                                                                                                                                                                                                                                                                                                                                                                                                                                                                                                                                                                                                                                                                                                                                                                                                                                                                                                                                                                                                                                                                                                                                                                                                                                                                                                                                                                                                                                                                                                                                                                                                                                                                                                                                                                                                                                                                                                                                                                                                                                                                                                                                                                                                                                                                                                                                                                                                                                                                                                                                                                       0,                                                                                                                                                                                                                                                                                                                                                                                                                                                                                                                                                                                                                                                                                                                                                                                                                                                                                                                                                                                                                                                                                                                                                                                                                                                                                                                                                                                                                                                                                                                                                                                                                                                                                                                                                                                                                                                                                                                                                                                                                                                                                                                                                                                                                                                                                                                                                                                                                                                                                                                                                                                                                                                                                                                                                                                                                                                                                                                                                                                                                                           -dq1*cos(q1),                                                                                                                                                                                                                                                                                                                                                                                                                                                                                                                                                                                                                                                                                                                                                                                                                                                                                                                                                                                                                                                                                                                                                                                                                                                                                                                                                                                                                                                                                                                                                                                                                                                                                                                                                                                                                                                                                                                                                                                                                                                                                                                                                                                                                                                                                                                                                                                                                                                                                                                                                                                                                                                                                                                                                                                                                                                                                                                                                                              dq1*cos(q1),                                                                                                                                                                                                                                                                                                                                                                                                                                                                                                                                                                                                                                                                                                                                                                                                                                                                                                                                                                                                                                                                                                                                                                                                                                                                                                                                                                                                                                                                                                                                                                                                                                                                                                                                                                                                                                                                                                                                                                                                                                                                                                                                                                                                                                                     dq2*cos(q1)*cos(q2)*cos(q3) - dq3*cos(q1)*cos(q2)*cos(q3) + dq1*cos(q2)*sin(q1)*sin(q3) - dq1*cos(q3)*sin(q1)*sin(q2) + dq2*cos(q1)*sin(q2)*sin(q3) - dq3*cos(q1)*sin(q2)*sin(q3),                                                                                                                                                                                                                                                                                                                                                                                                                                                                                                                                                                                                                                                                                                                                                                                                                                                                                                                                                                                                                                                                                                                                                                                                                                                                                                                                                                                                                                                                                                                                                                                                                                                                                                                                                                                                          (3^(1/2)*(sin(q4)*(dq1*cos(q2)*cos(q3)*sin(q1) - dq2*cos(q1)*cos(q2)*sin(q3) + dq2*cos(q1)*cos(q3)*sin(q2) + dq3*cos(q1)*cos(q2)*sin(q3) - dq3*cos(q1)*cos(q3)*sin(q2) + dq1*sin(q1)*sin(q2)*sin(q3)) - dq1*cos(q1)*cos(q4) + dq4*sin(q1)*sin(q4) - dq4*cos(q4)*(cos(q1)*cos(q2)*cos(q3) + cos(q1)*sin(q2)*sin(q3))))/2 + (dq2*cos(q1)*cos(q2)*cos(q3))/2 - (dq3*cos(q1)*cos(q2)*cos(q3))/2 + (dq1*cos(q2)*sin(q1)*sin(q3))/2 - (dq1*cos(q3)*sin(q1)*sin(q2))/2 + (dq2*cos(q1)*sin(q2)*sin(q3))/2 - (dq3*cos(q1)*sin(q2)*sin(q3))/2, (3^(1/2)*(sin(q4)*(dq1*cos(q2)*cos(q3)*sin(q1) - dq2*cos(q1)*cos(q2)*sin(q3) + dq2*cos(q1)*cos(q3)*sin(q2) + dq3*cos(q1)*cos(q2)*sin(q3) - dq3*cos(q1)*cos(q3)*sin(q2) + dq1*sin(q1)*sin(q2)*sin(q3)) - dq1*cos(q1)*cos(q4) + dq4*sin(q1)*sin(q4) - dq4*cos(q4)*(cos(q1)*cos(q2)*cos(q3) + cos(q1)*sin(q2)*sin(q3))))/4 - (3^(1/2)*((cos(q5)*(sin(q4)*(dq1*cos(q2)*cos(q3)*sin(q1) - dq2*cos(q1)*cos(q2)*sin(q3) + dq2*cos(q1)*cos(q3)*sin(q2) + dq3*cos(q1)*cos(q2)*sin(q3) - dq3*cos(q1)*cos(q3)*sin(q2) + dq1*sin(q1)*sin(q2)*sin(q3)) - dq1*cos(q1)*cos(q4) + dq4*sin(q1)*sin(q4) - dq4*cos(q4)*(cos(q1)*cos(q2)*cos(q3) + cos(q1)*sin(q2)*sin(q3))))/2 + sin(q5)*(cos(q4)*(dq1*cos(q2)*cos(q3)*sin(q1) - dq2*cos(q1)*cos(q2)*sin(q3) + dq2*cos(q1)*cos(q3)*sin(q2) + dq3*cos(q1)*cos(q2)*sin(q3) - dq3*cos(q1)*cos(q3)*sin(q2) + dq1*sin(q1)*sin(q2)*sin(q3)) + dq1*cos(q1)*sin(q4) + dq4*cos(q4)*sin(q1) + dq4*sin(q4)*(cos(q1)*cos(q2)*cos(q3) + cos(q1)*sin(q2)*sin(q3))) + dq5*cos(q5)*(sin(q1)*sin(q4) - cos(q4)*(cos(q1)*cos(q2)*cos(q3) + cos(q1)*sin(q2)*sin(q3))) + (dq5*sin(q5)*(cos(q4)*sin(q1) + sin(q4)*(cos(q1)*cos(q2)*cos(q3) + cos(q1)*sin(q2)*sin(q3))))/2 - (3^(1/2)*cos(q5)*(dq2*cos(q1)*cos(q2)*cos(q3) - dq3*cos(q1)*cos(q2)*cos(q3) + dq1*cos(q2)*sin(q1)*sin(q3) - dq1*cos(q3)*sin(q1)*sin(q2) + dq2*cos(q1)*sin(q2)*sin(q3) - dq3*cos(q1)*sin(q2)*sin(q3)))/2 - (3^(1/2)*dq5*sin(q5)*(cos(q1)*cos(q2)*sin(q3) - cos(q1)*cos(q3)*sin(q2)))/2))/2 + (dq2*cos(q1)*cos(q2)*cos(q3))/4 - (dq3*cos(q1)*cos(q2)*cos(q3))/4 + (dq1*cos(q2)*sin(q1)*sin(q3))/4 - (dq1*cos(q3)*sin(q1)*sin(q2))/4 + (dq2*cos(q1)*sin(q2)*sin(q3))/4 - (dq3*cos(q1)*sin(q2)*sin(q3))/4;
                                                                                                                                                                                                                                                                                                                                                                                                                                                                                                                                                                                                                                                                                                                                                                                                                                                                                                                                                                                                                                                                                                                                                                                                                                                                                                                                                                                                                                                                                                                                                                                                                                                                                                                                                                                                                                                                                                                                                                                                                                                                                                                                                                                                                                                                                                                                                                                                                                                                                                                                                                                                                                                                                                                                                                                                                                                                                                                                                                                                                                                                                                                                                                                                                                                                                                                                                                                       0,                                                                                                                                                                                                                                                                                                                                                                                                                                                                                                                                                                                                                                                                                                                                                                                                                                                                                                                                                                                                                                                                                                                                                                                                                                                                                                                                                                                                                                                                                                                                                                                                                                                                                                                                                                                                                                                                                                                                                                                                                                                                                                                                                                                                                                                                                                                                                                                                                                                                                                                                                                                                                                                                                                                                                                                                                                                                                                                                                                                                                                            dq1*sin(q1),                                                                                                                                                                                                                                                                                                                                                                                                                                                                                                                                                                                                                                                                                                                                                                                                                                                                                                                                                                                                                                                                                                                                                                                                                                                                                                                                                                                                                                                                                                                                                                                                                                                                                                                                                                                                                                                                                                                                                                                                                                                                                                                                                                                                                                                                                                                                                                                                                                                                                                                                                                                                                                                                                                                                                                                                                                                                                                                                                                             -dq1*sin(q1),                                                                                                                                                                                                                                                                                                                                                                                                                                                                                                                                                                                                                                                                                                                                                                                                                                                                                                                                                                                                                                                                                                                                                                                                                                                                                                                                                                                                                                                                                                                                                                                                                                                                                                                                                                                                                                                                                                                                                                                                                                                                                                                                                                                                                                                     dq1*cos(q1)*cos(q2)*sin(q3) - dq1*cos(q1)*cos(q3)*sin(q2) - dq2*cos(q2)*cos(q3)*sin(q1) + dq3*cos(q2)*cos(q3)*sin(q1) - dq2*sin(q1)*sin(q2)*sin(q3) + dq3*sin(q1)*sin(q2)*sin(q3),                                                                                                                                                                                                                                                                                                                                                                                                                                                                                                                                                                                                                                                                                                                                                                                                                                                                                                                                                                                                                                                                                                                                                                                                                                                                                                                                                                                                                                                                                                                                                                                                                                                                                                                                                                                                          (3^(1/2)*(sin(q4)*(dq1*cos(q1)*cos(q2)*cos(q3) + dq1*cos(q1)*sin(q2)*sin(q3) + dq2*cos(q2)*sin(q1)*sin(q3) - dq2*cos(q3)*sin(q1)*sin(q2) - dq3*cos(q2)*sin(q1)*sin(q3) + dq3*cos(q3)*sin(q1)*sin(q2)) + dq1*cos(q4)*sin(q1) + dq4*cos(q1)*sin(q4) + dq4*cos(q4)*(sin(q1)*sin(q2)*sin(q3) + cos(q2)*cos(q3)*sin(q1))))/2 + (dq1*cos(q1)*cos(q2)*sin(q3))/2 - (dq1*cos(q1)*cos(q3)*sin(q2))/2 - (dq2*cos(q2)*cos(q3)*sin(q1))/2 + (dq3*cos(q2)*cos(q3)*sin(q1))/2 - (dq2*sin(q1)*sin(q2)*sin(q3))/2 + (dq3*sin(q1)*sin(q2)*sin(q3))/2, (3^(1/2)*(sin(q4)*(dq1*cos(q1)*cos(q2)*cos(q3) + dq1*cos(q1)*sin(q2)*sin(q3) + dq2*cos(q2)*sin(q1)*sin(q3) - dq2*cos(q3)*sin(q1)*sin(q2) - dq3*cos(q2)*sin(q1)*sin(q3) + dq3*cos(q3)*sin(q1)*sin(q2)) + dq1*cos(q4)*sin(q1) + dq4*cos(q1)*sin(q4) + dq4*cos(q4)*(sin(q1)*sin(q2)*sin(q3) + cos(q2)*cos(q3)*sin(q1))))/4 - (3^(1/2)*((cos(q5)*(sin(q4)*(dq1*cos(q1)*cos(q2)*cos(q3) + dq1*cos(q1)*sin(q2)*sin(q3) + dq2*cos(q2)*sin(q1)*sin(q3) - dq2*cos(q3)*sin(q1)*sin(q2) - dq3*cos(q2)*sin(q1)*sin(q3) + dq3*cos(q3)*sin(q1)*sin(q2)) + dq1*cos(q4)*sin(q1) + dq4*cos(q1)*sin(q4) + dq4*cos(q4)*(sin(q1)*sin(q2)*sin(q3) + cos(q2)*cos(q3)*sin(q1))))/2 + sin(q5)*(cos(q4)*(dq1*cos(q1)*cos(q2)*cos(q3) + dq1*cos(q1)*sin(q2)*sin(q3) + dq2*cos(q2)*sin(q1)*sin(q3) - dq2*cos(q3)*sin(q1)*sin(q2) - dq3*cos(q2)*sin(q1)*sin(q3) + dq3*cos(q3)*sin(q1)*sin(q2)) - dq4*sin(q4)*(sin(q1)*sin(q2)*sin(q3) + cos(q2)*cos(q3)*sin(q1)) + dq4*cos(q1)*cos(q4) - dq1*sin(q1)*sin(q4)) - (3^(1/2)*cos(q5)*(dq1*cos(q1)*cos(q2)*sin(q3) - dq1*cos(q1)*cos(q3)*sin(q2) - dq2*cos(q2)*cos(q3)*sin(q1) + dq3*cos(q2)*cos(q3)*sin(q1) - dq2*sin(q1)*sin(q2)*sin(q3) + dq3*sin(q1)*sin(q2)*sin(q3)))/2 + dq5*cos(q5)*(cos(q1)*sin(q4) + cos(q4)*(sin(q1)*sin(q2)*sin(q3) + cos(q2)*cos(q3)*sin(q1))) + (dq5*sin(q5)*(cos(q1)*cos(q4) - sin(q4)*(sin(q1)*sin(q2)*sin(q3) + cos(q2)*cos(q3)*sin(q1))))/2 + (3^(1/2)*dq5*sin(q5)*(cos(q2)*sin(q1)*sin(q3) - cos(q3)*sin(q1)*sin(q2)))/2))/2 + (dq1*cos(q1)*cos(q2)*sin(q3))/4 - (dq1*cos(q1)*cos(q3)*sin(q2))/4 - (dq2*cos(q2)*cos(q3)*sin(q1))/4 + (dq3*cos(q2)*cos(q3)*sin(q1))/4 - (dq2*sin(q1)*sin(q2)*sin(q3))/4 + (dq3*sin(q1)*sin(q2)*sin(q3))/4;
                                                                                                                                                                                                                                                                                                                                                                                                                                                                                                                                                                                                                                                                                                                                                                                                                                                                                                                                                                                                                                                                                                                                                                                                                                                                                                                                                                                                                                                                                                                                                                                                                                                                                                                                                                                                                                                                                                                                                                                                                                                                                                                                                                                                                                                                                                                                                                                                                                                                                                                                                                                                                                                                                                                                                                                                                                                                                                                                                                                                                                                                                                                                                                                                                                                                                                                                                                                       0,                                                                                                                                                                                                                                                                                                                                                                                                                                                                                                                                                                                                                                                                                                                                                                                                                                                                                                                                                                                                                                                                                                                                                                                                                                                                                                                                                                                                                                                                                                                                                                                                                                                                                                                                                                                                                                                                                                                                                                                                                                                                                                                                                                                                                                                                                                                                                                                                                                                                                                                                                                                                                                                                                                                                                                                                                                                                                                                                                                                                                                                      0,                                                                                                                                                                                                                                                                                                                                                                                                                                                                                                                                                                                                                                                                                                                                                                                                                                                                                                                                                                                                                                                                                                                                                                                                                                                                                                                                                                                                                                                                                                                                                                                                                                                                                                                                                                                                                                                                                                                                                                                                                                                                                                                                                                                                                                                                                                                                                                                                                                                                                                                                                                                                                                                                                                                                                                                                                                                                                                                                                                                        0,                                                                                                                                                                                                                                                                                                                                                                                                                                                                                                                                                                                                                                                                                                                                                                                                                                                                                                                                                                                                                                                                                                                                                                                                                                                                                                                                                                                                                                                                                                                                                                                                                                                                                                                                                                                                                                                                                                                                                                                                                                                                                                                                                                                                                                                                                                                                                 dq2*cos(q3)*sin(q2) - dq2*cos(q2)*sin(q3) + dq3*cos(q2)*sin(q3) - dq3*cos(q3)*sin(q2),                                                                                                                                                                                                                                                                                                                                                                                                                                                                                                                                                                                                                                                                                                                                                                                                                                                                                                                                                                                                                                                                                                                                                                                                                                                                                                                                                                                                                                                                                                                                                                                                                                                                                                                                                                                                                                                                                                                                                                                                                                                            (dq2*cos(q3)*sin(q2))/2 - (dq2*cos(q2)*sin(q3))/2 + (dq3*cos(q2)*sin(q3))/2 - (dq3*cos(q3)*sin(q2))/2 - (3^(1/2)*sin(q4)*(dq2*cos(q2)*cos(q3) - dq3*cos(q2)*cos(q3) + dq2*sin(q2)*sin(q3) - dq3*sin(q2)*sin(q3)))/2 + (3^(1/2)*dq4*cos(q4)*(cos(q2)*sin(q3) - cos(q3)*sin(q2)))/2,                                                                                                                                                                                                                                                                                                                                                                                                                                                                                                                                                                                                                                                                                                                                       (3^(1/2)*(cos(q4)*sin(q5)*(dq2*cos(q2)*cos(q3) - dq3*cos(q2)*cos(q3) + dq2*sin(q2)*sin(q3) - dq3*sin(q2)*sin(q3)) + (cos(q5)*sin(q4)*(dq2*cos(q2)*cos(q3) - dq3*cos(q2)*cos(q3) + dq2*sin(q2)*sin(q3) - dq3*sin(q2)*sin(q3)))/2 - (3^(1/2)*cos(q5)*(dq2*cos(q2)*sin(q3) - dq2*cos(q3)*sin(q2) - dq3*cos(q2)*sin(q3) + dq3*cos(q3)*sin(q2)))/2 + dq4*sin(q4)*sin(q5)*(cos(q2)*sin(q3) - cos(q3)*sin(q2)) + (dq5*sin(q4)*sin(q5)*(cos(q2)*sin(q3) - cos(q3)*sin(q2)))/2 + (3^(1/2)*dq5*sin(q5)*(cos(q2)*cos(q3) + sin(q2)*sin(q3)))/2 - (dq4*cos(q4)*cos(q5)*(cos(q2)*sin(q3) - cos(q3)*sin(q2)))/2 - dq5*cos(q4)*cos(q5)*(cos(q2)*sin(q3) - cos(q3)*sin(q2))))/2 - (dq2*cos(q2)*sin(q3))/4 + (dq2*cos(q3)*sin(q2))/4 + (dq3*cos(q2)*sin(q3))/4 - (dq3*cos(q3)*sin(q2))/4 - (3^(1/2)*sin(q4)*(dq2*cos(q2)*cos(q3) - dq3*cos(q2)*cos(q3) + dq2*sin(q2)*sin(q3) - dq3*sin(q2)*sin(q3)))/4 + (3^(1/2)*dq4*cos(q4)*(cos(q2)*sin(q3) - cos(q3)*sin(q2)))/4];
   
%% Define the task space matrices
Hp=inv(transpose(jac))*H*inv(jac);
Cp=inv(transpose(jac))*C*inv(jac)-Hp*dJac*inv(jac);
Gp=inv(transpose(jac))*G;

%% Equivalent Task Space Vectors
p=[(29*cos(q1)*sin(q2))/100 - (7*sin(q1))/1000 + (37*cos(q4)*sin(q1))/1000 - (37*cos(q5)*(cos(q4)*sin(q1) + sin(q4)*(cos(q1)*cos(q2)*cos(q3) + cos(q1)*sin(q2)*sin(q3))))/2000 + (37*sin(q5)*(sin(q1)*sin(q4) - cos(q4)*(cos(q1)*cos(q2)*cos(q3) + cos(q1)*sin(q2)*sin(q3))))/1000 + (29*3^(1/2)*(sin(q5)*(sin(q1)*sin(q4) - cos(q4)*(cos(q1)*cos(q2)*cos(q3) + cos(q1)*sin(q2)*sin(q3))) - (cos(q5)*(cos(q4)*sin(q1) + sin(q4)*(cos(q1)*cos(q2)*cos(q3) + cos(q1)*sin(q2)*sin(q3))))/2 + (3^(1/2)*cos(q5)*(cos(q1)*cos(q2)*sin(q3) - cos(q1)*cos(q3)*sin(q2)))/2))/625 + (37*sin(q4)*(cos(q1)*cos(q2)*cos(q3) + cos(q1)*sin(q2)*sin(q3)))/1000 + (221*3^(1/2)*(cos(q4)*sin(q1) + sin(q4)*(cos(q1)*cos(q2)*cos(q3) + cos(q1)*sin(q2)*sin(q3))))/4000 + (37*3^(1/2)*cos(q5)*(cos(q1)*cos(q2)*sin(q3) - cos(q1)*cos(q3)*sin(q2)))/2000 + (4849*cos(q1)*cos(q2)*sin(q3))/20000 - (4849*cos(q1)*cos(q3)*sin(q2))/20000;
(37*cos(q1)*cos(q4))/1000 - (7*cos(q1))/1000 - (29*sin(q1)*sin(q2))/100 - (37*cos(q5)*(cos(q1)*cos(q4) - sin(q4)*(sin(q1)*sin(q2)*sin(q3) + cos(q2)*cos(q3)*sin(q1))))/2000 + (37*sin(q5)*(cos(q1)*sin(q4) + cos(q4)*(sin(q1)*sin(q2)*sin(q3) + cos(q2)*cos(q3)*sin(q1))))/1000 - (29*3^(1/2)*((cos(q5)*(cos(q1)*cos(q4) - sin(q4)*(sin(q1)*sin(q2)*sin(q3) + cos(q2)*cos(q3)*sin(q1))))/2 - sin(q5)*(cos(q1)*sin(q4) + cos(q4)*(sin(q1)*sin(q2)*sin(q3) + cos(q2)*cos(q3)*sin(q1))) + (3^(1/2)*cos(q5)*(cos(q2)*sin(q1)*sin(q3) - cos(q3)*sin(q1)*sin(q2)))/2))/625 - (37*sin(q4)*(sin(q1)*sin(q2)*sin(q3) + cos(q2)*cos(q3)*sin(q1)))/1000 + (221*3^(1/2)*(cos(q1)*cos(q4) - sin(q4)*(sin(q1)*sin(q2)*sin(q3) + cos(q2)*cos(q3)*sin(q1))))/4000 - (37*3^(1/2)*cos(q5)*(cos(q2)*sin(q1)*sin(q3) - cos(q3)*sin(q1)*sin(q2)))/2000 - (4849*cos(q2)*sin(q1)*sin(q3))/20000 + (4849*cos(q3)*sin(q1)*sin(q2))/20000;
                                                                                                                                                                                                                                                                                                (4849*cos(q2)*cos(q3))/20000 - (29*cos(q2))/100 + (4849*sin(q2)*sin(q3))/20000 + (29*3^(1/2)*((3^(1/2)*cos(q5)*(cos(q2)*cos(q3) + sin(q2)*sin(q3)))/2 + cos(q4)*sin(q5)*(cos(q2)*sin(q3) - cos(q3)*sin(q2)) + (cos(q5)*sin(q4)*(cos(q2)*sin(q3) - cos(q3)*sin(q2)))/2))/625 - (37*sin(q4)*(cos(q2)*sin(q3) - cos(q3)*sin(q2)))/1000 + (37*3^(1/2)*cos(q5)*(cos(q2)*cos(q3) + sin(q2)*sin(q3)))/2000 - (221*3^(1/2)*sin(q4)*(cos(q2)*sin(q3) - cos(q3)*sin(q2)))/4000 + (37*cos(q4)*sin(q5)*(cos(q2)*sin(q3) - cos(q3)*sin(q2)))/1000 + (37*cos(q5)*sin(q4)*(cos(q2)*sin(q3) - cos(q3)*sin(q2)))/2000 + 689/2500;
0;
0;
0];
 
pd=[(29*cos(qd1)*sin(qd2))/100 - (7*sin(qd1))/1000 + (37*cos(qd4)*sin(qd1))/1000 - (37*cos(qd5)*(cos(qd4)*sin(qd1) + sin(qd4)*(cos(qd1)*cos(qd2)*cos(qd3) + cos(qd1)*sin(qd2)*sin(qd3))))/2000 + (37*sin(qd5)*(sin(qd1)*sin(qd4) - cos(qd4)*(cos(qd1)*cos(qd2)*cos(qd3) + cos(qd1)*sin(qd2)*sin(qd3))))/1000 + (29*3^(1/2)*(sin(qd5)*(sin(qd1)*sin(qd4) - cos(qd4)*(cos(qd1)*cos(qd2)*cos(qd3) + cos(qd1)*sin(qd2)*sin(qd3))) - (cos(qd5)*(cos(qd4)*sin(qd1) + sin(qd4)*(cos(qd1)*cos(qd2)*cos(qd3) + cos(qd1)*sin(qd2)*sin(qd3))))/2 + (3^(1/2)*cos(qd5)*(cos(qd1)*cos(qd2)*sin(qd3) - cos(qd1)*cos(qd3)*sin(qd2)))/2))/625 + (37*sin(qd4)*(cos(qd1)*cos(qd2)*cos(qd3) + cos(qd1)*sin(qd2)*sin(qd3)))/1000 + (221*3^(1/2)*(cos(qd4)*sin(qd1) + sin(qd4)*(cos(qd1)*cos(qd2)*cos(qd3) + cos(qd1)*sin(qd2)*sin(qd3))))/4000 + (37*3^(1/2)*cos(qd5)*(cos(qd1)*cos(qd2)*sin(qd3) - cos(qd1)*cos(qd3)*sin(qd2)))/2000 + (4849*cos(qd1)*cos(qd2)*sin(qd3))/20000 - (4849*cos(qd1)*cos(qd3)*sin(qd2))/20000;
(37*cos(qd1)*cos(qd4))/1000 - (7*cos(qd1))/1000 - (29*sin(qd1)*sin(qd2))/100 - (37*cos(qd5)*(cos(qd1)*cos(qd4) - sin(qd4)*(sin(qd1)*sin(qd2)*sin(qd3) + cos(qd2)*cos(qd3)*sin(qd1))))/2000 + (37*sin(qd5)*(cos(qd1)*sin(qd4) + cos(qd4)*(sin(qd1)*sin(qd2)*sin(qd3) + cos(qd2)*cos(qd3)*sin(qd1))))/1000 - (29*3^(1/2)*((cos(qd5)*(cos(qd1)*cos(qd4) - sin(qd4)*(sin(qd1)*sin(qd2)*sin(qd3) + cos(qd2)*cos(qd3)*sin(qd1))))/2 - sin(qd5)*(cos(qd1)*sin(qd4) + cos(qd4)*(sin(qd1)*sin(qd2)*sin(qd3) + cos(qd2)*cos(qd3)*sin(qd1))) + (3^(1/2)*cos(qd5)*(cos(qd2)*sin(qd1)*sin(qd3) - cos(qd3)*sin(qd1)*sin(qd2)))/2))/625 - (37*sin(qd4)*(sin(qd1)*sin(qd2)*sin(qd3) + cos(qd2)*cos(qd3)*sin(qd1)))/1000 + (221*3^(1/2)*(cos(qd1)*cos(qd4) - sin(qd4)*(sin(qd1)*sin(qd2)*sin(qd3) + cos(qd2)*cos(qd3)*sin(qd1))))/4000 - (37*3^(1/2)*cos(qd5)*(cos(qd2)*sin(qd1)*sin(qd3) - cos(qd3)*sin(qd1)*sin(qd2)))/2000 - (4849*cos(qd2)*sin(qd1)*sin(qd3))/20000 + (4849*cos(qd3)*sin(qd1)*sin(qd2))/20000;
                                                                                                                                                                                                                                                                                                                                (4849*cos(qd2)*cos(qd3))/20000 - (29*cos(qd2))/100 + (4849*sin(qd2)*sin(qd3))/20000 + (29*3^(1/2)*((3^(1/2)*cos(qd5)*(cos(qd2)*cos(qd3) + sin(qd2)*sin(qd3)))/2 + cos(qd4)*sin(qd5)*(cos(qd2)*sin(qd3) - cos(qd3)*sin(qd2)) + (cos(qd5)*sin(qd4)*(cos(qd2)*sin(qd3) - cos(qd3)*sin(qd2)))/2))/625 - (37*sin(qd4)*(cos(qd2)*sin(qd3) - cos(qd3)*sin(qd2)))/1000 + (37*3^(1/2)*cos(qd5)*(cos(qd2)*cos(qd3) + sin(qd2)*sin(qd3)))/2000 - (221*3^(1/2)*sin(qd4)*(cos(qd2)*sin(qd3) - cos(qd3)*sin(qd2)))/4000 + (37*cos(qd4)*sin(qd5)*(cos(qd2)*sin(qd3) - cos(qd3)*sin(qd2)))/1000 + (37*cos(qd5)*sin(qd4)*(cos(qd2)*sin(qd3) - cos(qd3)*sin(qd2)))/2000 + 689/2500;
0;
0;
0];                                                                                                                                                                                                                                                                                                                                
 
dp=jac*dq;
dpd=jac*dqd;

% ddp=jac*ddq+dJac*dq;
ddpd=jac*ddqd+dJac*dqd;
                                 
%% Function output
%Define the stiffness and damping matrix below for task space directions
Km=70*eye(6);
Dm=50*eye(6);
Hm=2*eye(6);

jacT=transpose(jac);
u0=ddpd+inv(Hm)*(Dm*(dpd-dp)+Km*(pd-p)+f);
torque=G+25*(qd-q)+0*jacT*(Hp*u0+Cp*dp+Gp-f);
test=pd-p;
